simulink model "GFo_29bus"  (R2017b)
settings: Solver=ode1  StartTime=0.0  StopTime=4.5  FixedStep=Time_Step  RelTol=1e-3  EnableMultiTasking=on
PreLoadFcn:
  | Init_29bus;
InitFcn:
  | Init_29bus;
undefined symbols (not defined in the file): D1, D11, Delta, Time_Step, VSC01_Delta_P_Time_Step, VSC01_Delta_P_Value
libraries: powerlib x169, sps_avr x6, GFo_Lib x1
(part 2 of 5)

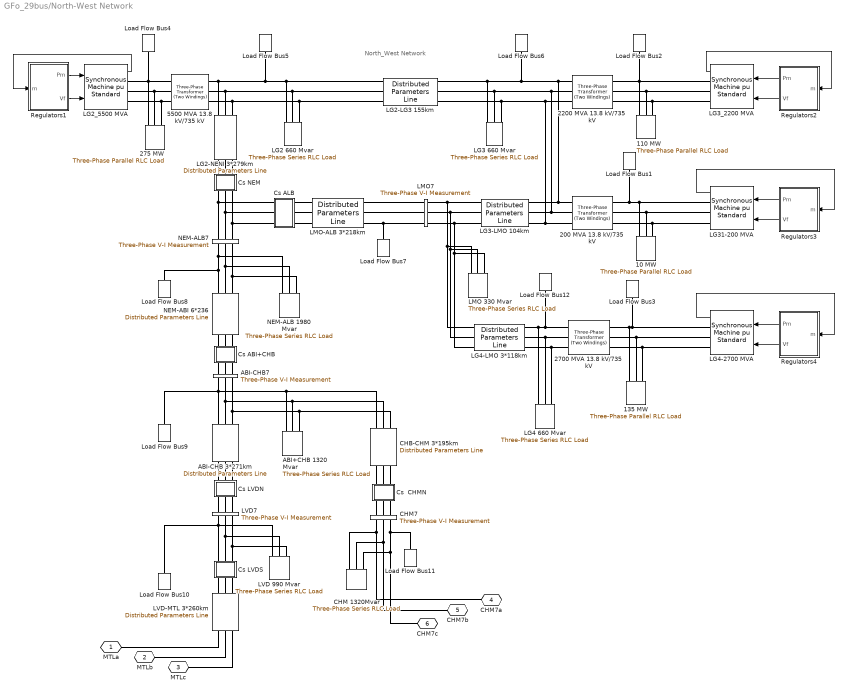
== system GFo_29bus/North-West Network ==
  note: North_West Network
  10 MW : powerlib/Elements/Three-Phase Parallel RLC Load  LConnTagsString=A|B|C  Configuration=Y (grounded)  NominalVoltage=(13800)*1  Vabc=[1e3 1e3 1e3]  Vabcp=[1e3 1e3 1e3]  NominalFrequency=60  UnbalancedPower=off  ActivePower=10000000  InductivePower=0  CapacitivePower=0  Pabc=[10e3 9e3 11e3]  QLabc=[100 90 110]  QCabc=[100 90 110]  Pabcp=[10e3 9e3 11e3]  QLabcp=[100 90 110]  QCabcp=[100 90 110]  Measurements=None  LoadType=constant PQ
  110 MW : powerlib/Elements/Three-Phase Parallel RLC Load  LConnTagsString=A|B|C  Configuration=Y (grounded)  NominalVoltage=(13800)*1  Vabc=[1e3 1e3 1e3]  Vabcp=[1e3 1e3 1e3]  NominalFrequency=60  UnbalancedPower=off  ActivePower=110000000  InductivePower=0  CapacitivePower=0  Pabc=[10e3 9e3 11e3]  QLabc=[100 90 110]  QCabc=[100 90 110]  Pabcp=[10e3 9e3 11e3]  QLabcp=[100 90 110]  QCabcp=[100 90 110]  Measurements=None  LoadType=constant PQ
  135 MW : powerlib/Elements/Three-Phase Parallel RLC Load  LConnTagsString=A|B|C  Configuration=Y (grounded)  NominalVoltage=(13800)*1  Vabc=[1e3 1e3 1e3]  Vabcp=[1e3 1e3 1e3]  NominalFrequency=60  UnbalancedPower=off  ActivePower=135000000  InductivePower=0  CapacitivePower=0  Pabc=[10e3 9e3 11e3]  QLabc=[100 90 110]  QCabc=[100 90 110]  Pabcp=[10e3 9e3 11e3]  QLabcp=[100 90 110]  QCabcp=[100 90 110]  Measurements=None  LoadType=constant PQ
  200 MVA 13.8 kV/735 kV : powerlib/Elements/Three-Phase Transformer (Two Windings)  Winding1Connection=Delta (D1)  Winding2Connection=Yg  CoreType=Three single-phase transformers  SetSaturation=off  Hysteresis=off  DataFile='basic_model'  SetInitialFlux=off  Measurements=None  UNITS=pu  NominalPower=[ 200e6 60 ]  Winding1="[ 13.8e3 0.002  0.0]"  Winding2=[ 735e3 0.002 0.12]  Rm=500  Lm=500  L0=0.5  Saturation="[ 0,0  ;  0.005,1.2  ;  1.0,1.4 ]"  InitialFluxes=[ 0.8 , -0.8 , 0.7 ]  BreakLoop=off  DiscreteSolver=Trapezoidal iterative  DataType=off  TransfoNumber=0
  2200 MVA 13.8 kV/735 kV : powerlib/Elements/Three-Phase Transformer (Two Windings)  Winding1Connection=Delta (D1)  Winding2Connection=Yg  CoreType=Three single-phase transformers  SetSaturation=off  Hysteresis=off  DataFile='basic_model'  SetInitialFlux=off  Measurements=None  UNITS=pu  NominalPower=[ 2200e6 60 ]  Winding1="[ 13.8e3 0.002  0.0]"  Winding2=[ 735e3 0.002 0.12]  Rm=500  Lm=500  L0=0.5  Saturation="[ 0,0  ;  0.005,1.2  ;  1.0,1.4 ]"  InitialFluxes=[ 0.8 , -0.8 , 0.7 ]  BreakLoop=off  DiscreteSolver=Trapezoidal iterative  DataType=off  TransfoNumber=0
  2700 MVA 13.8 kV/735 kV : powerlib/Elements/Three-Phase Transformer (Two Windings)  Winding1Connection=Delta (D1)  Winding2Connection=Yg  CoreType=Three single-phase transformers  SetSaturation=off  Hysteresis=off  DataFile='basic_model'  SetInitialFlux=off  Measurements=None  UNITS=pu  NominalPower=[ 2700e6 60 ]  Winding1="[ 13.8e3 0.002  0.0]"  Winding2=[ 735e3 0.002 0.12]  Rm=500  Lm=500  L0=0.5  Saturation="[ 0,0  ;  0.005,1.2  ;  1.0,1.4 ]"  InitialFluxes=[ 0.8 , -0.8 , 0.7 ]  BreakLoop=off  DiscreteSolver=Trapezoidal iterative  DataType=off  TransfoNumber=0
  275 MW : powerlib/Elements/Three-Phase Parallel RLC Load  LConnTagsString=A|B|C  Configuration=Y (grounded)  NominalVoltage=(13800)*1  Vabc=[1e3 1e3 1e3]  Vabcp=[1e3 1e3 1e3]  NominalFrequency=60  UnbalancedPower=off  ActivePower=275000000  InductivePower=0  CapacitivePower=0  Pabc=[10e3 9e3 11e3]  QLabc=[100 90 110]  QCabc=[100 90 110]  Pabcp=[10e3 9e3 11e3]  QLabcp=[100 90 110]  QCabcp=[100 90 110]  Measurements=None  LoadType=constant PQ
  5500 MVA 13.8 kV/735 kV : powerlib/Elements/Three-Phase Transformer (Two Windings)  Winding1Connection=Delta (D1)  Winding2Connection=Yg  CoreType=Three single-phase transformers  SetSaturation=off  Hysteresis=off  DataFile='basic_model'  SetInitialFlux=off  Measurements=None  UNITS=pu  NominalPower=[ 5500e6 60 ]  Winding1="[ 13.8e3 0.002  0.0]"  Winding2=[ 735e3 0.002 0.12]  Rm=500  Lm=500  L0=0.5  Saturation="[ 0,0  ;  0.005,1.2  ;  1.0,1.4 ]"  InitialFluxes=[ 0.8 , -0.8 , 0.7 ]  BreakLoop=off  DiscreteSolver=Trapezoidal iterative  DataType=off  TransfoNumber=0
  ABI+CHB 1320 Mvar : powerlib/Elements/Three-Phase Series RLC Load  LConnTagsString=A|B|C  Configuration=Y (grounded)  NominalVoltage=735e3  Vabc=[1e3 1e3 1e3]  Vabcp=[1e3 1e3 1e3]  NominalFrequency=60  UnbalancedPower=off  ActivePower=4400000  InductivePower=1320e6  CapacitivePower=0  Pabc=[10e3 9e3 11e3]  QLabc=[100 90 110]  QCabc=[100 90 110]  Pabcp=[10e3 9e3 11e3]  QLabcp=[100 90 110]  QCabcp=[100 90 110]  Measurements=None  LoadType=constant Z
  ABI-CHB 3*271km : powerlib/Elements/Distributed Parameters Line  Phases=3  Length=271  Frequency=60  Resistance="[0.01273  0.3864]/3"  Inductance="[0.9337e-3  4.1264e-3]/3"  Capacitance=[12.74e-9 7.751e-9]*3  x1=[-0.00156 -4.29903868088888e-08 0 0;-0.00152 -4.31049710047087e-08 0 0;-0.00148 -4.32097535018435e-08 0 0;-0.00144 -4.33047104736571e-08 0 0;-0.0014 -4.33898203277529e-08 0 0;-0.00136 -4.34650637108841e-08 0 0;-0.00132 -4.35304235133541e-08 0 0;-0.00128 -4.35858848729076e-08 0 0;-0.00124 -4.36314351781097e-08 0 0;-0.0012 -4.36670640712137e-08 0 0;-0.00116 -4.36927634505166e-08 0 0;-0.00112 -4.37085274722013e-08 0 0;-0.00108 -4.3714352551665e-08 0 0;-0.00104 -4.37102373643351e-08 0 0;-0.001 -4.36961828459695e-08 0 0;-0.00096 -4.36721921924446e-08 187826.147216155 -755236.018624265;-0.00092 -4.3638270859028e-08 199193.07837854 -752317.887920411;-0.00088 -4.35944265591385e-08 210514.71475267 -749228.686616557;-0.00084 -4.35406692625918e-08 221788.481896066 -745969.117170439;-0.0008 -4.34770111933336e-08 233011.816251302 -742539.920780041;-0.00076 -4.34034668266597e-08 244182.16572893 -738941.877215048;-0.00072 -4.3320052885925e-08 255296.99028781 -735175.804639541;-0.00068 -4.32267883387403e-08 266353.762512685 -731242.559425944;-0.00064 -4.31236943926593e-08 277349.968188901 -727143.035960301;-0.0006 -4.30107944903563e-08 288283.106874116 -722878.166438896;-0.00056 -4.28881143042955e-08 299150.692466876 -718448.920656278;-0.00052 -4.27556817308933e-08 309950.253771934 -713856.305784742;-0.00048 -4.26135268841747e-08 320679.335062181 -709101.366145305;-0.00044 -4.24616820889261e-08 331335.496637056 -704185.182970237;-0.0004 -4.23001818733444e-08 341916.315377312 -699108.874157196;-0.00036 -4.2129062961186e-08 352419.385296011 -693873.594015029;-0.00032 -4.19483642634157e-08 362842.318085629 -688480.533001295;-0.00028 -4.17581268693592e-08 373182.743661134 -682930.917451559;-0.00024 -4.15583940373594e-08 383438.310698921 -677226.00930054;-0.0002 -4.13492111849398e-08 393606.687171486 -671367.105795155;-0.00016 -4.11306258784772e-08 403685.560877708 -665355.539199535;-0.00012 -4.09026878223852e-08 413672.639968623 -659192.676492083;-8e-05 -4.06654488478122e-08 423565.653468569 -652879.919054632;-4e-05 -4.0418962900855e-08 433362.351791591 -646418.702353785]  x2=[-0.00156 -9.05659079389774e-08 0 0;-0.00152 -9.07557342875418e-08 0 0;-0.00148 -9.09249235647733e-08 0 0;-0.00144 -9.10734372984894e-08 0 0;-0.0014 -9.12012417179476e-08 0 0;-0.00136 -9.13083077615252e-08 0 0;-0.00132 -9.13946110833272e-08 0 0;-0.00128 -9.14601320587224e-08 0 0;-0.00124 -9.15048557888059e-08 0 0;-0.0012 -9.15287721037874e-08 0 0;-0.00116 -9.1531875565303e-08 0 0;-0.00112 -9.15141654676524e-08 0 0;-0.00108 -9.14756458379589e-08 0 0;-0.00104 -9.14163254352542e-08 0 0;-0.001 -9.13362177484864e-08 0 0;-0.00096 -9.12353409934526e-08 -41952.3785132872 -761003.958676694;-0.00092 -9.11137181086569e-08 -30472.3572703532 -761550.015312388;-0.00088 -9.09713767500946e-08 -18985.4068761582 -761922.902041928;-0.00084 -9.08083492849631e-08 -7494.13936416284 -762122.534074088;-0.0008 -9.0624672784302e-08 3998.83225049725 -762148.866014263;-0.00076 -9.04203890145636e-08 15490.8945651881 -762001.891874799;-0.00072 -9.01955444281156e-08 26979.4343840425 -761681.645076347;-0.00068 -8.99501901526778e-08 38461.8393121788 -761188.198440267;-0.00064 -8.96843819796967e-08 49935.4983497363 -760521.664172069;-0.0006 -8.93981803516586e-08 61397.8024855944 -759682.193835898;-0.00056 -8.90916503483457e-08 72846.1452906394 -758669.97832007;-0.00052 -8.87648616720371e-08 84277.9235104437 -757485.247793662;-0.00048 -8.84178886316599e-08 95690.5376572236 -756128.271654181;-0.00044 -8.80508101258913e-08 107081.39260094 -754599.358466298;-0.0004 -8.76637096252179e-08 118447.89815941 -752898.855891687;-0.00036 -8.72566751529554e-08 129787.46968729 -751027.15060997;-0.00032 -8.68297992652326e-08 141097.528663802 -748984.668230786;-0.00028 -8.63831790299452e-08 152375.503279069 -746771.873197016;-0.00024 -8.59169160046831e-08 163618.829018921 -744389.268679167;-0.0002 -8.54311162136376e-08 174824.949248043 -741837.39646096;-0.00016 -8.49258901234916e-08 185991.315791332 -739116.836816131;-0.00012 -8.44013526183013e-08 197115.38951333 -736228.208376482;-8e-05 -8.38576229733718e-08 208194.640895605 -733172.16799121;-4e-05 -8.32948248281354e-08 219226.550611933 -729949.410577544]  x3=[-0.00156 -1.87807393079567e-10 0 0;-0.00152 -1.93846462957491e-10 0 0;-0.00148 -1.998414538214e-10 0 0;-0.00144 -2.05791002462069e-10 0 0;-0.0014 -2.11693756003443e-10 0 0;-0.00136 -2.17548372210272e-10 0 0;-0.00132 -2.23353519793318e-10 0 0;-0.00128 -2.29107878712081e-10 0 0;-0.00124 -2.34810140474967e-10 0 0;-0.0012 -2.40459008436826e-10 0 0;-0.00116 -2.46053198093796e-10 0 0;-0.00112 -2.51591437375393e-10 0 0;-0.00108 -2.57072466933762e-10 0 0;-0.00104 -2.62495040430049e-10 0 0;-0.001 -2.67857924817803e-10 0 0;-0.00096 -2.73159900623362e-10 139.26170460855 -1341.51413253579;-0.00092 -2.78399762223149e-10 159.474777343631 -1339.26171709775;-0.00088 -2.83576318117825e-10 179.651586889596 -1336.70476509455;-0.00084 -2.88688391203218e-10 199.787545213952 -1333.84385795502;-0.0008 -2.93734819037995e-10 219.87807357342 -1330.67964622477;-0.00076 -2.98714454107983e-10 239.918603555106 -1327.21284941825;-0.00072 -3.03626164087111e-10 259.904578115313 -1323.44425585518;-0.00068 -3.08468832094887e-10 279.831452615779 -1319.37472248122;-0.00064 -3.13241356950365e-10 299.694695857083 -1315.00517467318;-0.0006 -3.17942653422552e-10 319.489791109006 -1310.33660602853;-0.00056 -3.22571652477171e-10 339.212237137594 -1305.37007813954;-0.00052 -3.27127301519756e-10 358.857549228699 -1300.10672035181;-0.00048 -3.31608564635002e-10 378.421260207764 -1294.54772950751;-0.00044 -3.36014422822319e-10 397.898921455624 -1288.69436967323;-0.0004 -3.40343874227552e-10 417.28610392008 -1282.54797185251;-0.00036 -3.44595934370786e-10 436.578399123026 -1276.10993368321;-0.00032 -3.48769636370213e-10 455.771420162903 -1269.3817191197;-0.00028 -3.52864031161991e-10 474.86080271224 -1262.36485809994;-0.00024 -3.56878187716052e-10 493.842206010066 -1255.06094619762;-0.0002 -3.60811193247813e-10 512.711313848959 -1247.47164425932;-0.00016 -3.64662153425733e-10 531.463835556517 -1239.59867802686;-0.00012 -3.68430192574676e-10 550.095506971018 -1231.44383774485;-8e-05 -3.72114453875034e-10 568.602091411056 -1223.00897775366;-4e-05 -3.7571409955756e-10 586.979380638922 -1214.29601606771]  x4=[-0.00156 -2.85151300335962e-10 0 0;-0.00152 -2.82558887702488e-10 0 0;-0.00148 -2.79902223614635e-10 0 0;-0.00144 -2.77181912174905e-10 0 0;-0.0014 -2.74398571958662e-10 0 0;-0.00136 -2.71552835873468e-10 0 0;-0.00132 -2.68645351015168e-10 0 0;-0.00128 -2.65676778520747e-10 0 0;-0.00124 -2.62647793417989e-10 0 0;-0.0012 -2.59559084471985e-10 0 0;-0.00116 -2.56411354028515e-10 0 0;-0.00112 -2.53205317854336e-10 0 0;-0.00108 -2.49941704974427e-10 0 0;-0.00104 -2.46621257506212e-10 0 0;-0.001 -2.43244730490811e-10 0 0;-0.00096 -2.3981289172135e-10 -1510.55195138726 -15585.3803111079;-0.00092 -2.36326521568369e-10 -1275.36683491832 -15606.38544091;-0.00088 -2.32786412802377e-10 -1039.89171102942 -15623.8418132467;-0.00084 -2.29193370413579e-10 -804.180124733081 -15637.7454586893;-0.0008 -2.25548211428828e-10 -568.285674811329 -15648.0932156687;-0.00076 -2.21851764725842e-10 -332.262001627809 -15654.8827311943;-0.00072 -2.18104870844727e-10 -96.1627749304264 -15658.1124613888;-0.00068 -2.14308381796837e-10 139.958318352703 -15657.7816718394;-0.00064 -2.10463160871044e-10 376.047586321189 -15653.8904377648;-0.0006 -2.06570082437426e-10 612.051344311441 -15646.439643998;-0.00056 -2.02630031748445e-10 847.915927104103 -15635.4309847854;-0.00052 -1.98643904737653e-10 1083.58770112706 -15620.866963401;-0.00048 -1.94612607815955e-10 1319.01307665124 -15602.7508915777;-0.00044 -1.90537057665507e-10 1554.13851997647 -15581.0868887541;-0.0004 -1.86418181031268e-10 1788.91056560458 -15555.8798811376;-0.00036 -1.82256914510264e-10 2023.27582839698 -15527.1356005843;-0.00032 -1.78054204338617e-10 2257.18101571399 -15494.8605832957;-0.00028 -1.73811006176378e-10 2490.57293953313 -15459.0621683325;-0.00024 -1.69528284890216e-10 2723.3985285436 -15419.7484959455;-0.0002 -1.6520701433402e-10 2955.60484021427 -15376.9285057247;-0.00016 -1.60848177127449e-10 3187.13907283233 -15330.6119345667;-0.00012 -1.56452764432495e-10 3417.94857750994 -15280.8093144604;-8e-05 -1.520217757281e-10 3647.98087015616 -15227.531970092;-4e-05 -1.47556218582885e-10 3877.18364341136 -15170.7920162703]  x5=0.00153261764655846  V1=ones(3,3)  V2=ones(3,3)  I1=ones(3,3)  I2=ones(3,3)  nHarmo=1  Measurements=None  Decoupling=off  VsMag0=0  VrMag0=0  VsAngle0=0  VrAngle0=0  IsMag0=0  IrMag0=0  IsAngle0=0  IrAngle0=0
      settings: AttributesFormatString=\n
  ABI-CHB7 : powerlib/Measurements/Three-Phase V-I Measurement  VoltageMeasurement=no  SetLabelV=on  LabelV=Vabc_ABI7  Vpu=on  VpuLL=off  CurrentMeasurement=no  SetLabelI=off  LabelI=A1  Ipu=off  Pbase=100e6  Vbase=500e3  OutputType=Magnitude  PhasorSimulation=off  PSBequivalent=0
  CHB-CHM 3*195km : powerlib/Elements/Distributed Parameters Line  Phases=3  Length=195  Frequency=60  Resistance="[0.01273  0.3864]/3"  Inductance="[0.9337e-3  4.1264e-3]/3"  Capacitance=[12.74e-9 7.751e-9]*3  x1=[-0.00112 -4.32880028151544e-08 0 0;-0.00108 -4.32972814037169e-08 0 0;-0.00104 -4.32967145638679e-08 0 0;-0.001 -4.32863024245021e-08 0 0;-0.00096 -4.32660473532502e-08 0 0;-0.00092 -4.32359539559406e-08 0 0;-0.00088 -4.31960290755524e-08 0 0;-0.00084 -4.31462817906592e-08 0 0;-0.0008 -4.30867234133644e-08 0 0;-0.00076 -4.30173674867295e-08 0 0;-0.00072 -4.29382297816941e-08 0 0;-0.00068 -4.28493282934899e-08 266353.762512684 -731242.559425945;-0.00064 -4.27506832375486e-08 277349.968188901 -727143.035960302;-0.0006 -4.26423170449053e-08 288283.106874116 -722878.166438896;-0.00056 -4.25242543570976e-08 299150.692466875 -718448.920656278;-0.00052 -4.23965220205627e-08 309950.253771933 -713856.305784743;-0.00048 -4.22591490805323e-08 320679.335062181 -709101.366145306;-0.00044 -4.21121667744285e-08 331335.496637056 -704185.182970238;-0.0004 -4.19556085247599e-08 341916.315377311 -699108.874157197;-0.00036 -4.17895099315226e-08 352419.385296011 -693873.59401503;-0.00032 -4.16139087641043e-08 362842.318085629 -688480.533001296;-0.00028 -4.1428844952696e-08 373182.743661134 -682930.91745156;-0.00024 -4.12343605792127e-08 383438.310698921 -677226.009300541;-0.0002 -4.10304998677236e-08 393606.687171486 -671367.105795156;-0.00016 -4.08173091743966e-08 403685.560877708 -665355.539199536;-0.00012 -4.05948369769568e-08 413672.639968622 -659192.676492084;-8e-05 -4.03631338636634e-08 423565.653468569 -652879.919054633;-4e-05 -4.01222525218062e-08 433362.351791591 -646418.702353786]  x2=[-0.00112 -3.01476576023589e-08 0 0;-0.00108 -3.01218550239861e-08 0 0;-0.00104 -3.00892029955408e-08 0 0;-0.001 -3.00497089418125e-08 0 0;-0.00096 -3.00033818434085e-08 0 0;-0.00092 -2.99502322347114e-08 0 0;-0.00088 -2.9890272201484e-08 0 0;-0.00084 -2.98235153781207e-08 0 0;-0.0008 -2.97499769445474e-08 0 0;-0.00076 -2.96696736227698e-08 0 0;-0.00072 -2.95826236730708e-08 0 0;-0.00068 -2.94888468898582e-08 189059.279164108 -739106.876621136;-0.00064 -2.93883645971639e-08 200182.856377785 -736171.980404537;-0.0006 -2.92811996437946e-08 211260.913736226 -733069.685028072;-0.00056 -2.91673763981366e-08 222290.93218472 -729800.695926955;-0.00052 -2.90469207426144e-08 233270.40359219 -726365.756441117;-0.00048 -2.89198600678053e-08 244196.831321521 -722765.647646176;-0.00044 -2.87862232662111e-08 255067.730797274 -719001.188175825;-0.0004 -2.86460407256879e-08 265880.630070654 -715073.234035686;-0.00036 -2.84993443225366e-08 276633.070381613 -710982.678408656;-0.00032 -2.83461674142543e-08 287322.606717949 -706730.451451809;-0.00028 -2.81865448319489e-08 297946.808371282 -702317.520084886;-0.00024 -2.80205128724192e-08 308503.259489775 -697744.887770424;-0.0002 -2.78481092899009e-08 318989.559627479 -693013.594285579;-0.00016 -2.76693732874819e-08 329403.324290172 -688124.715485687;-0.00012 -2.74843455081878e-08 339742.185477576 -683079.36305963;-8e-05 -2.72930680257401e-08 350003.792221813 -677878.684277038;-4e-05 -2.70955843349887e-08 360185.811122003 -672523.861727418]  x3=[-0.00112 -1.55990618873976e-10 0 0;-0.00108 -1.5474156304947e-10 0 0;-0.00104 -1.5345732032796e-10 0 0;-0.001 -1.52138182735167e-10 0 0;-0.00096 -1.50784450231604e-10 0 0;-0.00092 -1.49396430644368e-10 0 0;-0.00088 -1.47974439597144e-10 0 0;-0.00084 -1.46518800438432e-10 0 0;-0.0008 -1.45029844168025e-10 0 0;-0.00076 -1.43507909361738e-10 0 0;-0.00072 -1.41953342094422e-10 0 0;-0.00068 -1.40366495861267e-10 1436.68883540973 -5039.584986483;-0.00064 -1.38747731497423e-10 1512.51770857072 -5017.34797479882;-0.0006 -1.37097417095945e-10 1588.00264824819 -4993.97006145294;-0.00056 -1.35415927924098e-10 1663.1264898178 -4969.45656238125;-0.00052 -1.33703646338018e-10 1737.87215076581 -4943.81305174204;-0.00048 -1.31960961695771e-10 1812.22263457351 -4917.04536064849;-0.00044 -1.30188270268818e-10 1886.16103458205 -4889.15957584272;-0.0004 -1.28385975151902e-10 1959.67053783689 -4860.16203831173;-0.00036 -1.26554486171389e-10 2032.7344289109 -4830.05934184547;-0.00032 -1.24694219792081e-10 2105.33609370534 -4798.85833153754;-0.00028 -1.22805599022509e-10 2177.45902322771 -4766.56610222861;-0.00024 -1.2088905331875e-10 2249.0868173458 -4733.18999689314;-0.0002 -1.18945018486769e-10 2320.20318851693 -4698.73760496967;-0.00016 -1.16973936583322e-10 2390.79196549157 -4663.21676063503;-0.00012 -1.14976255815436e-10 2460.83709699057 -4626.63554102288;-8e-05 -1.12952430438491e-10 2530.32265535507 -4589.00226438711;-4e-05 -1.10902920652924e-10 2599.23284016831 -4550.32548821028]  x4=[-0.00112 -1.20875953871152e-10 0 0;-0.00108 -1.23066019964183e-10 0 0;-0.00104 -1.25228101905551e-10 0 0;-0.001 -1.27361708056466e-10 0 0;-0.00096 -1.2946635325329e-10 0 0;-0.00092 -1.31541558917854e-10 0 0;-0.00088 -1.33586853166286e-10 0 0;-0.00084 -1.35601770916312e-10 0 0;-0.0008 -1.37585853993012e-10 0 0;-0.00076 -1.39538651233004e-10 0 0;-0.00072 -1.41459718587035e-10 0 0;-0.00068 -1.43348619220956e-10 1508.00651437468 -11782.2938614793;-0.00064 -1.45204923615053e-10 1685.50172841821 -11758.214496796;-0.0006 -1.47028209661713e-10 1862.61367390384 -11731.4614155346;-0.00056 -1.48818062761413e-10 2039.30207710253 -11702.0407011152;-0.00052 -1.50574075916994e-10 2215.52676059507 -11669.9590435544;-0.00048 -1.52295849826207e-10 2391.24765240814 -11635.2237379446;-0.00044 -1.53982992972513e-10 2566.4247951263 -11597.8426827946;-0.0004 -1.55635121714109e-10 2741.01835497795 -11557.8243782342;-0.00036 -1.57251860371168e-10 2914.98863089321 -11515.1779240805;-0.00032 -1.58832841311261e-10 3088.2960635316 -11469.9130177696;-0.00028 -1.60377705032956e-10 3260.90124427747 -11422.0399521507;-0.00024 -1.61886100247564e-10 3432.76492420121 -11371.5696131462;-0.0002 -1.63357683959023e-10 3603.84802298409 -11318.513477276;-0.00016 -1.64792121541886e-10 3774.1116378048 -11262.8836090476;-0.00012 -1.66189086817417e-10 3943.51705218563 -11204.6926582136;-8e-05 -1.67548262127759e-10 4112.02574479624 -11143.9538568943;-4e-05 -1.68869338408169e-10 4279.59939821308 -11080.6810165692]  x5=0.0011028060556417  V1=ones(3,3)  V2=ones(3,3)  I1=ones(3,3)  I2=ones(3,3)  nHarmo=1  Measurements=None  Decoupling=off  VsMag0=0  VrMag0=0  VsAngle0=0  VrAngle0=0  IsMag0=0  IrMag0=0  IsAngle0=0  IrAngle0=0
      settings: AttributesFormatString=\n
  CHM 1320Mvar : powerlib/Elements/Three-Phase Series RLC Load  LConnTagsString=A|B|C  Configuration=Y (grounded)  NominalVoltage=735e3  Vabc=[1e3 1e3 1e3]  Vabcp=[1e3 1e3 1e3]  NominalFrequency=60  UnbalancedPower=off  ActivePower=4400000  InductivePower=1320e6  CapacitivePower=0  Pabc=[10e3 9e3 11e3]  QLabc=[100 90 110]  QCabc=[100 90 110]  Pabcp=[10e3 9e3 11e3]  QLabcp=[100 90 110]  QCabcp=[100 90 110]  Measurements=None  LoadType=constant Z
  CHM7 : powerlib/Measurements/Three-Phase V-I Measurement  VoltageMeasurement=no  SetLabelV=on  LabelV=Vabc_CHM7  Vpu=on  VpuLL=off  CurrentMeasurement=no  SetLabelI=off  LabelI=A1  Ipu=off  Pbase=100e6  Vbase=735e3  OutputType=Magnitude  PhasorSimulation=off  PSBequivalent=0
  "Cs  CHMN " : Subsystem  mask{Xc=25/3}
      mask prompts: Xc "Condensator Reactance at  60Hz  (ohm):"
      mask help: Series Compensation
      mask init:
      | Cs=1/Xc/(2*pi*60);
      mask Display: disp('Cs')
  "Cs ABI+CHB " : Subsystem  mask{Xc=25/6}
      mask prompts: Xc "Condensator Reactance at  60Hz  (ohm):"
      mask help: Series Compensation
      mask init:
      | Cs=1/Xc/(2*pi*60);
      mask Display: disp('Cs')
  Cs ALB : Subsystem  mask{Xc=16/3}
      mask prompts: Xc "Reactance @ 60Hz du condensateur (ohm):"
      mask init:
      | Cs=1/Xc/(2*pi*60);
      mask Display: disp('Cs')
  "Cs LVDN " : Subsystem  mask{Xc=34/3}
      mask prompts: Xc "Condensator Reactance at  60Hz  (ohm):"
      mask help: Series Compensation
      mask init:
      | Cs=1/Xc/(2*pi*60);
      mask Display: disp('Cs')
  "Cs LVDS " : Subsystem  mask{Xc=34/3}
      mask prompts: Xc "Condensator Reactance at  60Hz  (ohm):"
      mask help: Series Compensation
      mask init:
      | Cs=1/Xc/(2*pi*60);
      mask Display: disp('Cs')
  "Cs NEM " : Subsystem  mask{Xc=16/3}
      mask prompts: Xc "Condensator Reactance at  60Hz  (ohm):"
      mask help: Series Compensation
      mask init:
      | Cs=1/Xc/(2*pi*60);
      mask Display: disp('Cs')
  LG2 660 Mvar : powerlib/Elements/Three-Phase Series RLC Load  LConnTagsString=A|B|C  Configuration=Y (grounded)  NominalVoltage=735e3  Vabc=[1e3 1e3 1e3]  Vabcp=[1e3 1e3 1e3]  NominalFrequency=60  UnbalancedPower=off  ActivePower=2200000  InductivePower=660e6  CapacitivePower=0  Pabc=[10e3 9e3 11e3]  QLabc=[100 90 110]  QCabc=[100 90 110]  Pabcp=[10e3 9e3 11e3]  QLabcp=[100 90 110]  QCabcp=[100 90 110]  Measurements=None  LoadType=constant Z
  LG2-LG3 155km : powerlib/Elements/Distributed Parameters Line  Phases=3  Length=155  Frequency=60  Resistance="[0.01273  0.3864]"  Inductance="[0.9337e-3  4.1264e-3]"  Capacitance=[12.74e-9 7.751e-9]  x1=[-0.00088 -2.79013421874721e-09 432972.643007631 -601762.460463105;-0.00084 -2.80512262966329e-09 441997.469610389 -595165.210789451;-0.0008 -2.81947317988372e-09 450921.789800182 -588432.625679351;-0.00076 -2.83318260621716e-09 459743.574263559 -581566.236064597;-0.00072 -2.84624779125826e-09 468460.817002808 -574567.603302976;-0.00068 -2.85866576409663e-09 477071.535792104 -567438.318823225;-0.00064 -2.87043370099233e-09 485573.772628251 -560180.003763152;-0.0006 -2.88154892601799e-09 493965.594175912 -552794.30860101;-0.00056 -2.89200891166729e-09 502245.092207235 -545282.912780187;-0.00052 -2.9018112794297e-09 510410.384035767 -537647.524327318;-0.00048 -2.91095380033132e-09 518459.612944562 -529889.879463891;-0.00044 -2.91943439544175e-09 526390.948608378 -522011.742211451;-0.0004 -2.92725113634678e-09 534202.587509883 -514014.903990468;-0.00036 -2.93440224558694e-09 541892.753349755 -505901.183212994;-0.00032 -2.94088609706166e-09 549459.697450599 -497672.424869164;-0.00028 -2.94670121639904e-09 556901.699154582 -489330.500107662;-0.00024 -2.95184628129107e-09 564217.066214693 -480877.305810242;-0.0002 -2.95632012179438e-09 571404.135179547 -472314.764160391;-0.00016 -2.96012172059621e-09 578461.271771641 -463644.822206238;-0.00012 -2.96325021324578e-09 585386.871258971 -454869.451417819;-8e-05 -2.96570488835083e-09 592179.358819939 -445990.647238774;-4e-05 -2.96748518773943e-09 598837.189901448 -437010.428632606]  x2=[-0.00088 -1.73659978268186e-09 445028.99986202 -584528.468417321;-0.00084 -1.75470646929317e-09 453792.58140898 -577751.376044598;-0.0008 -1.77241415078531e-09 462452.974436268 -570842.907991278;-0.00076 -1.78971880058422e-09 471008.209645194 -563804.635183421;-0.00072 -1.80661648376174e-09 479456.341649048 -556638.158063567;-0.00068 -1.82310335793046e-09 487795.449415467 -549345.106226812;-0.00064 -1.83917567411735e-09 496023.636703258 -541927.138050252;-0.0006 -1.85482977761633e-09 504139.032493588 -534385.94031588;-0.00056 -1.87006210881925e-09 512139.791415439 -526723.227827028;-0.00052 -1.88486920402535e-09 520024.094165227 -518940.743018436;-0.00048 -1.89924769622888e-09 527790.147920499 -511040.255560035;-0.00044 -1.9131943158847e-09 535436.186747602 -503023.561954544;-0.0004 -1.92670589165177e-09 542960.472003244 -494892.485128955;-0.00036 -1.93977935111428e-09 550361.292729844 -486648.874020019;-0.00032 -1.95241172148029e-09 557636.96604459 -478294.603153812;-0.00028 -1.96460013025773e-09 564785.837522115 -469831.572219484;-0.00024 -1.97634180590753e-09 571806.281570693 -461261.705637289;-0.0002 -1.98763407847391e-09 578696.701801889 -452586.952120983;-0.00016 -1.99847438019147e-09 585455.531393563 -443809.284234708;-0.00012 -2.00886024606909e-09 592081.233446151 -434930.697944447;-8e-05 -2.01878931445043e-09 598572.301332146 -425953.212164156;-4e-05 -2.02825932755095e-09 604927.259038684 -416878.868296683]  x3=[-0.00088 -1.84558852963393e-12 1691.06014924484 -2581.83555987813;-0.00084 -1.82016083348527e-12 1729.79962719175 -2556.042391552;-0.0008 -1.79431924845947e-12 1768.1457636206 -2529.66800122839;-0.00076 -1.76806965071012e-12 1806.08983895064 -2502.71838621624;-0.00072 -1.74141800916939e-12 1843.62322502635 -2475.19967462559;-0.00068 -1.71437038419072e-12 1880.73738707943 -2447.11812397413;-0.00064 -1.68693292617078e-12 1917.42388566947 -2418.48011976434;-0.0006 -1.65911187415093e-12 1953.67437860307 -2389.29217403139;-0.00056 -1.63091355439846e-12 1989.48062283075 -2359.56092386245;-0.00052 -1.60234437896812e-12 2024.83447632134 -2329.29312988741;-0.00048 -1.57341084424404e-12 2059.72789991345 -2298.4956747416;-0.00044 -1.54411952946249e-12 2094.15295914345 -2267.17556150074;-0.0004 -1.51447709521586e-12 2128.10182604975 -2235.33991208848;-0.00036 -1.48449028193807e-12 2161.56678095278 -2202.99596565696;-0.00032 -1.45416590837187e-12 2194.54021421037 -2170.15107694068;-0.00028 -1.4235108700183e-12 2227.01462794816 -2136.81271458409;-0.00024 -1.39253213756872e-12 2258.98263776451 -2102.98845944329;-0.0002 -1.36123675531974e-12 2290.43697440968 -2068.68600286221;-0.00016 -1.32963183957141e-12 2321.37048543874 -2033.91314492367;-0.00012 -1.29772457700902e-12 2351.77613683807 -1998.6777926757;-8e-05 -1.26552222306891e-12 2381.64701462473 -1962.98795833353;-4e-05 -1.23303210028868e-12 2410.97632641872 -1926.85175745773]  x4=[-0.00088 -4.62619871537164e-12 1092.96989342995 -2102.93040181752;-0.00084 -4.72627398977189e-12 1124.55604688283 -2086.21026082643;-0.0008 -4.82527455022451e-12 1155.8864859884 -2069.01573361274;-0.00076 -4.92317788485581e-12 1186.95408647501 -2051.35073006366;-0.00072 -5.01996173129177e-12 1217.7517838382 -2033.21926704865;-0.00068 -5.11560408172034e-12 1248.2725749472 -2014.62546750606;-0.00064 -5.21008318789582e-12 1278.50951963729 -1995.57355950554;-0.0006 -5.30337756608421e-12 1308.45574228802 -1976.06787528669;-0.00056 -5.39546600194846e-12 1338.10443338659 -1956.11285027387;-0.00052 -5.48632755537238e-12 1367.44885107633 -1935.71302206771;-0.00048 -5.57594156522228e-12 1396.48232268971 -1914.8730294132;-0.00044 -5.66428765404513e-12 1425.19824626567 -1893.59761114497;-0.0004 -5.75134573270218e-12 1453.59009205081 -1871.89160510966;-0.00036 -5.83709600493711e-12 1481.65140398424 -1849.75994706585;-0.00032 -5.92151897187748e-12 1509.37580116563 -1827.20766956172;-0.00028 -6.00459543646866e-12 1536.75697930613 -1804.23990079071;-0.00024 -6.08630650783901e-12 1563.78871216196 -1780.86186342535;-0.0002 -6.16663360559555e-12 1590.46485295019 -1757.07887342976;-0.00016 -6.24555846404895e-12 1616.77933574645 -1732.89633885075;-0.00012 -6.32306313636704e-12 1642.72617686427 -1708.31975858814;-8e-05 -6.39912999865569e-12 1668.29947621573 -1683.35472114436;-4e-05 -6.4737417539664e-12 1693.49341865311 -1658.00690335361]  x5=0.000876589428843401  V1=ones(3,3)  V2=ones(3,3)  I1=ones(3,3)  I2=ones(3,3)  nHarmo=1  Measurements=None  Decoupling=off  VsMag0=0  VrMag0=0  VsAngle0=0  VrAngle0=0  IsMag0=0  IrMag0=0  IsAngle0=0  IrAngle0=0
      settings: AttributesFormatString=\n
  LG2-NENI 3*279km : powerlib/Elements/Distributed Parameters Line  Phases=3  Length=279  Frequency=60  Resistance="[0.01273  0.3864]/3"  Inductance="[0.9337e-3  4.1264e-3]/3"  Capacitance=[12.74e-9 7.751e-9]*3  x1=[-0.0016 -2.41583924208325e-09 0 0;-0.00156 -2.4415900454317e-09 0 0;-0.00152 -2.46678565225921e-09 0 0;-0.00148 -2.49142033330204e-09 0 0;-0.00144 -2.51548848684617e-09 0 0;-0.0014 -2.53898464000105e-09 0 0;-0.00136 -2.56190344994405e-09 0 0;-0.00132 -2.58423970513546e-09 0 0;-0.00128 -2.60598832650345e-09 0 0;-0.00124 -2.62714436859908e-09 0 0;-0.0012 -2.64770302072082e-09 0 0;-0.00116 -2.66765960800847e-09 0 0;-0.00112 -2.68700959250617e-09 0 0;-0.00108 -2.70574857419432e-09 0 0;-0.00104 -2.72387229199008e-09 0 0;-0.001 -2.74137662471631e-09 405315.757865484 -620727.351198764;-0.00096 -2.75825759203871e-09 414629.701621834 -614544.98398557;-0.00092 -2.77451135537088e-09 423849.362159649 -608222.874542627;-0.00088 -2.79013421874721e-09 432972.643007631 -601762.460463105;-0.00084 -2.80512262966329e-09 441997.469610389 -595165.210789451;-0.0008 -2.81947317988372e-09 450921.789800182 -588432.625679351;-0.00076 -2.83318260621716e-09 459743.574263559 -581566.236064597;-0.00072 -2.84624779125826e-09 468460.817002808 -574567.603302976;-0.00068 -2.85866576409663e-09 477071.535792104 -567438.318823225;-0.00064 -2.87043370099233e-09 485573.772628251 -560180.003763152;-0.0006 -2.88154892601799e-09 493965.594175912 -552794.30860101;-0.00056 -2.89200891166729e-09 502245.092207235 -545282.912780187;-0.00052 -2.9018112794297e-09 510410.384035767 -537647.524327318;-0.00048 -2.91095380033132e-09 518459.612944562 -529889.879463891;-0.00044 -2.91943439544175e-09 526390.948608378 -522011.742211451;-0.0004 -2.92725113634678e-09 534202.587509883 -514014.903990468;-0.00036 -2.93440224558694e-09 541892.753349755 -505901.183212994;-0.00032 -2.94088609706166e-09 549459.697450599 -497672.424869164;-0.00028 -2.94670121639904e-09 556901.699154582 -489330.500107662;-0.00024 -2.95184628129107e-09 564217.066214693 -480877.305810242;-0.0002 -2.95632012179438e-09 571404.135179547 -472314.764160391;-0.00016 -2.96012172059621e-09 578461.271771641 -463644.822206238;-0.00012 -2.96325021324578e-09 585386.871258971 -454869.451417819;-8e-05 -2.96570488835083e-09 592179.358819939 -445990.647238774;-4e-05 -2.96748518773943e-09 598837.189901448 -437010.428632606]  x2=[-0.0016 -2.65953235838337e-08 0 0;-0.00156 -2.66692370020041e-08 0 0;-0.00152 -2.6737086065666e-08 0 0;-0.00148 -2.67988553465273e-08 0 0;-0.00144 -2.68545307987864e-08 0 0;-0.0014 -2.69040997623254e-08 0 0;-0.00136 -2.69475509655895e-08 0 0;-0.00132 -2.69848745281498e-08 0 0;-0.00128 -2.70160619629501e-08 0 0;-0.00124 -2.70411061782365e-08 0 0;-0.0012 -2.70600014791707e-08 0 0;-0.00116 -2.70727435691239e-08 0 0;-0.00112 -2.7079329550655e-08 0 0;-0.00108 -2.70797579261684e-08 0 0;-0.00104 -2.70740285982553e-08 0 0;-0.001 -2.70621428697155e-08 243862.200065526 -727663.308973734;-0.00096 -2.7044103443261e-08 254806.991474596 -723903.345217305;-0.00092 -2.7019914420902e-08 265693.841971167 -719978.77208285;-0.00088 -2.69895813030134e-08 276520.27597932 -715890.481984456;-0.00084 -2.69531109870848e-08 287283.831661325 -711639.404564035;-0.0008 -2.69105117661515e-08 297982.06147744 -707226.506479933;-0.00076 -2.68617933269089e-08 308612.532742463 -702652.79118712;-0.00072 -2.680696674751e-08 319172.828178901 -697919.29870901;-0.00068 -2.67460444950462e-08 329660.54646664 -693027.105400973;-0.00064 -2.66790404227122e-08 340073.302788985 -687977.323705579;-0.0006 -2.66059697666564e-08 350408.729374943 -682771.101899639;-0.00056 -2.65268491425158e-08 360664.476037637 -677409.623833093;-0.00052 -2.64416965416379e-08 370838.210708718 -671894.10865982;-0.00048 -2.635053132699e-08 380927.619968656 -666225.810560406;-0.00044 -2.62533742287556e-08 390930.409572794 -660406.018456956;-0.0004 -2.6150247339621e-08 400844.304973034 -654436.055720009;-0.00036 -2.60411741097515e-08 410667.051835058 -648317.279867607;-0.00032 -2.59261793414591e-08 420396.416550937 -642051.082256614;-0.00028 -2.58052891835622e-08 430030.186747036 -635638.887766327;-0.00024 -2.56785311254403e-08 439566.171787091 -629082.15447448;-0.0002 -2.55459339907826e-08 449002.203270339 -622382.373325678;-0.00016 -2.54075279310343e-08 458336.135524594 -615541.067792378;-0.00012 -2.52633444185396e-08 467565.846094152 -608559.793528464;-8e-05 -2.51134162393859e-08 476689.236222426 -601440.138015496;-4e-05 -2.49577774859483e-08 485704.231329174 -594183.720201743]  x3=[-0.0016 -1.94345070726738e-11 0 0;-0.00156 -2.20044197367152e-11 0 0;-0.00152 -2.45693287854664e-11 0 0;-0.00148 -2.71286509807287e-11 0 0;-0.00144 -2.96818043547055e-11 0 0;-0.0014 -3.2228208342337e-11 0 0;-0.00136 -3.47672839133157e-11 0 0;-0.00132 -3.72984537037529e-11 0 0;-0.00128 -3.98211421474659e-11 0 0;-0.00124 -4.23347756068575e-11 0 0;-0.0012 -4.48387825033557e-11 0 0;-0.00116 -4.73325934473858e-11 0 0;-0.00112 -4.98156413678448e-11 0 0;-0.00108 -5.22873616410486e-11 0 0;-0.00104 -5.47471922191222e-11 0 0;-0.001 -5.7194573757805e-11 -295.463539845799 -2742.88515404389;-0.00096 -5.96289497436401e-11 -254.069695761354 -2747.02858680455;-0.00092 -6.20497666205217e-11 -212.618078419097 -2750.54736895394;-0.00088 -6.44564739155682e-11 -171.118113559348 -2753.44070035133;-0.00084 -6.68485243642953e-11 -129.579237916235 -2755.70792307813;-0.0008 -6.9225374035059e-11 -88.0108970718639 -2757.34852158744;-0.00076 -7.15864824527414e-11 -46.4225433084721 -2758.3621228213;-0.00072 -7.39313127216495e-11 -4.823633459063 -2758.74849629552;-0.00068 -7.62593316476013e-11 36.7763732429975 -2758.50755415213;-0.00064 -7.85700098591688e-11 78.3680173149285 -2757.63935117928;-0.0006 -8.08628219280533e-11 119.941841175539 -2756.14408479883;-0.00056 -8.31372464885626e-11 161.488391295801 -2754.02209502148;-0.00052 -8.53927663561655e-11 202.998220348498 -2751.2738643694;-0.00048 -8.76288686450949e-11 244.461889356471 -2747.90001776653;-0.00044 -8.98450448849735e-11 285.869969838953 -2743.9013223965;-0.0004 -9.2040791136436e-11 327.213045955531 -2739.27868752816;-0.00036 -9.421560810572e-11 368.481716647225 -2734.03316430881;-0.00032 -9.63690012582015e-11 409.666597774204 -2728.16594552519;-0.00028 -9.85004809308479e-11 450.758324249663 -2721.67836533226;-0.00024 -1.00609562443563e-10 491.747552169362 -2714.57189894981;-0.0002 -1.02695766209397e-10 532.624960936348 -2706.84816232701;-0.00016 -1.04758617843607e-10 573.381255380379 -2698.50891177496;-0.00012 -1.06797648271518e-10 614.007167871566 -2689.55604356732;-8e-05 -1.08812393835197e-10 654.493460427751 -2679.99159350911;-4e-05 -1.10802396398875e-10 694.830926815146 -2669.81773647381]  x4=[-0.0016 -7.71465364255446e-11 0 0;-0.00156 -7.54489471332153e-11 0 0;-0.00152 -7.37342014009519e-11 0 0;-0.00148 -7.20026891471466e-11 0 0;-0.00144 -7.02548041027539e-11 0 0;-0.0014 -6.849094372176e-11 0 0;-0.00136 -6.67115090908044e-11 0 0;-0.00132 -6.49169048379772e-11 0 0;-0.00128 -6.31075390408094e-11 0 0;-0.00124 -6.12838231334798e-11 0 0;-0.0012 -5.9446171813259e-11 0 0;-0.00116 -5.75950029462097e-11 0 0;-0.00112 -5.57307374721687e-11 0 0;-0.00108 -5.38537993090279e-11 0 0;-0.00104 -5.19646152563396e-11 0 0;-0.001 -5.00636148982657e-11 4695.72941749421 -13362.2957077408;-0.00096 -4.81512305058942e-11 4896.68712230303 -13289.9688778721;-0.00092 -4.62278969389442e-11 5096.53136268747 -13214.6200236884;-0.00088 -4.42940515468827e-11 5295.21669579065 -13136.2662788693;-0.00084 -4.23501340694751e-11 5492.69794228121 -13054.9254603807;-0.0008 -4.0396586536792e-11 5688.93019662671 -12970.6160644233;-0.00076 -3.84338531686959e-11 5883.86883730474 -12883.3572622267;-0.00072 -3.64623802738286e-11 6077.46953694948 -12793.1688956901;-0.00068 -3.44826161481252e-11 6269.68827243139 -12700.0714728701;-0.00064 -3.24950109728751e-11 6460.48133486764 -12604.0861633179;-0.0006 -3.05000167123548e-11 6649.80533956116 -12505.2347932652;-0.00056 -2.84980870110551e-11 6837.61723586594 -12403.5398406611;-0.00052 -2.64896770905262e-11 7023.87431697638 -12299.0244300608;-0.00048 -2.4475243645864e-11 7208.53422963846 -12191.7123273674;-0.00044 -2.24552447418623e-11 7391.55498378047 -12081.6279344275;-0.0004 -2.04301397088522e-11 7572.89496206122 -11968.7962834829;-0.00036 -1.84003890382542e-11 7752.51292933346 -11853.243031478;-0.00032 -1.63664542778671e-11 7930.3680420204 -11734.9944542257;-0.00028 -1.43287979269155e-11 8106.41985740317 -11614.0774404328;-0.00024 -1.22878833308817e-11 8280.62834281714 -11490.5194855854;-0.0002 -1.02441745761446e-11 8452.95388475506 -11364.3486856971;-0.00016 -8.19813638445086e-12 8623.35729787476 -11235.5937309196;-0.00012 -6.15023400724103e-12 8791.79983390958 -11104.2838990193;-8e-05 -4.10093311985532e-12 8958.24319047943 -10970.4490487197;-4e-05 -2.05069971564309e-12 9122.64951980036 -10834.1196129115]  x5=0.00157786097191812  V1=ones(3,3)  V2=ones(3,3)  I1=ones(3,3)  I2=ones(3,3)  nHarmo=1  Measurements=None  Decoupling=off  VsMag0=0  VrMag0=0  VsAngle0=0  VrAngle0=0  IsMag0=0  IrMag0=0  IsAngle0=0  IrAngle0=0
      settings: AttributesFormatString=\n
  LG2_5500 MVA : powerlib/Machines/Synchronous Machine pu Standard  PresetModel=No  MechanicalLoad=Mechanical power Pm  ShowDetailedParameters=on  RotorType=Salient-pole  Units=per unit standard parameters  MeasurementBus=off  NominalParameters="[5500E6  13800   60 ]"  Reactances1=[ 31 32 33 34 35 36 37 ]  Reactances2=[ 1.305, 0.296, 0.252, 0.474, 0.243, 0.18 ]  dAxisTimeConstants=Short-circuit  qAxisTimeConstants=Open-circuit  TimeConstants1=[]  TimeConstants2=[]  TimeConstants3=[]  TimeConstants4=[]  TimeConstants5=[ 1.01, 0.053, 0.1 ]  TimeConstants6=[]  TimeConstants7=[]  TimeConstants8=[]  StatorResistance=2.8544e-3  Mechanical="[ 4.1  0  32]"  PolePairs=32  InitialConditions=[0 -68.2322 0.822292 0.822292 0.822292 4.1842 -115.816 124.184 1.25511]  SetSaturation=off  Saturation=[0.6404,0.7127,0.8441,0.9214,0.9956,1.082,1.19,1.316,1.457;0.7,0.7698,0.8872,0.9466,0.9969,1.046,1.1,1.151,1.201]  LoadFlowParameters=[2 4000000000 0 0 0]  TsPowergui=0  TsBlock=-1  IterativeModel=Trapezoidal non iterative  IterativeDiscreteModel=Trapezoidal non iterative  BusType=swing  Pref=0  Qref=0  Qmin=-Inf  Qmax=Inf  PLF=0  QLF=0
      settings: AttributesFormatString=\n\n
  LG3 660 Mvar : powerlib/Elements/Three-Phase Series RLC Load  LConnTagsString=A|B|C  Configuration=Y (grounded)  NominalVoltage=735e3  Vabc=[1e3 1e3 1e3]  Vabcp=[1e3 1e3 1e3]  NominalFrequency=60  UnbalancedPower=off  ActivePower=2200000  InductivePower=660e6  CapacitivePower=0  Pabc=[10e3 9e3 11e3]  QLabc=[100 90 110]  QCabc=[100 90 110]  Pabcp=[10e3 9e3 11e3]  QLabcp=[100 90 110]  QCabcp=[100 90 110]  Measurements=None  LoadType=constant Z
  LG3-LMO 104km : powerlib/Elements/Distributed Parameters Line  Phases=3  Length=104  Frequency=60  Resistance="[0.01273  0.3864]"  Inductance="[0.9337e-3  4.1264e-3]"  Capacitance=[12.74e-9 7.751e-9]  x1=[-0.0006 -1.84830263941326e-09 0 0;-0.00056 -1.86396339240874e-09 0 0;-0.00052 -1.87920029620293e-09 0 0;-0.00048 -1.89400988605529e-09 0 0;-0.00044 -1.90838879439281e-09 0 0;-0.0004 -1.92233375157573e-09 0 0;-0.00036 -1.93584158664104e-09 550361.292729844 -486648.874020019;-0.00032 -1.94890922802354e-09 557636.96604459 -478294.603153812;-0.00028 -1.96153370425426e-09 564785.837522115 -469831.572219484;-0.00024 -1.97371214463618e-09 571806.281570693 -461261.705637289;-0.0002 -1.98544177989698e-09 578696.701801889 -452586.952120983;-0.00016 -1.99671994281875e-09 585455.531393563 -443809.284234708;-0.00012 -2.0075440688445e-09 592081.233446151 -434930.697944447;-8e-05 -2.01791169666132e-09 598572.301332146 -425953.212164156;-4e-05 -2.02782046876005e-09 604927.259038684 -416878.868296683]  x2=[-0.0006 -1.03652618900468e-08 0 0;-0.00056 -1.03424105982859e-08 0 0;-0.00052 -1.03172075315441e-08 0 0;-0.00048 -1.02896584207814e-08 0 0;-0.00044 -1.0259769530428e-08 0 0;-0.0004 -1.022754765696e-08 0 0;-0.00036 -1.01930001273533e-08 509416.858098534 -556033.052302243;-0.00032 -1.01561347974184e-08 517743.436837333 -548288.300411814;-0.00028 -1.01169600500133e-08 525952.285183424 -540418.872490108;-0.00024 -1.00754847931378e-08 534041.536515484 -532426.557977173;-0.0002 -1.00317184579076e-08 542009.351407518 -524313.174256404;-0.00016 -9.98567099640994e-09 549853.918047132 -516080.566241293;-0.00012 -9.93735287944046e-09 557573.45264752 -507730.605955909;-8e-05 -9.88677509412227e-09 565166.199853084 -499265.192109212;-4e-05 -9.83394914140759e-09 572630.433138588 -490686.249663309]  x3=[-0.0006 -2.5891516730553e-11 0 0;-0.00056 -2.65642269247652e-11 0 0;-0.00052 -2.72308966428549e-11 0 0;-0.00048 -2.78913742898772e-11 0 0;-0.00044 -2.8545509678911e-11 0 0;-0.0004 -2.91931540652098e-11 0 0;-0.00036 -2.98341601800252e-11 -30.215477134681 -878.894027383642;-0.00032 -3.04683822640945e-11 -16.958916126324 -879.249677062614;-0.00028 -3.10956761007851e-11 -3.69849880668731 -879.405392947349;-0.00024 -3.1715899048888e-11 9.5627595196835 -879.361139629396;-0.0002 -3.23289100750535e-11 22.8218433570053 -879.116927171579;-0.00016 -3.29345697858606e-11 36.0757377039548 -878.672811105705;-0.00012 -3.3532740459514e-11 49.3214287392544 -878.028892419937;-8e-05 -3.4123286077161e-11 62.5559045069886 -877.185317535831;-4e-05 -3.47060723538207e-11 75.7761556014971 -876.142278275042]  x4=[-0.0006 1.25600763098792e-11 0 0;-0.00056 1.32080406000832e-11 0 0;-0.00052 1.3853001495756e-11 0 0;-0.00048 1.44948123383518e-11 0 0;-0.00044 1.51333271856198e-11 0 0;-0.0004 1.57684008447901e-11 0 0;-0.00036 1.63998889055892e-11 3670.37159989901 -3222.94831504442;-0.00032 1.70276477730778e-11 3718.55339649164 -3167.23609882145;-0.00028 1.76515347003029e-11 3765.88962610934 -3110.80368042269;-0.00024 1.82714078207575e-11 3812.36952490171 -3053.66389209344;-0.0002 1.88871261806397e-11 3857.98252374059 -2995.82972692879;-0.00016 1.94985497709039e-11 3902.7182506234 -2937.31433591918;-0.00012 2.01055395590986e-11 3946.56653303163 -2878.13102495989;-8e-05 2.07079575209804e-11 3989.51740024398 -2818.29325182548;-4e-05 2.13056666718997e-11 4031.56108560365 -2757.81462310953]  x5=0.000588163229675572  V1=ones(3,3)  V2=ones(3,3)  I1=ones(3,3)  I2=ones(3,3)  nHarmo=1  Measurements=None  Decoupling=off  VsMag0=0  VrMag0=0  VsAngle0=0  VrAngle0=0  IsMag0=0  IrMag0=0  IsAngle0=0  IrAngle0=0
      settings: AttributesFormatString=\n
  LG31-200 MVA : powerlib/Machines/Synchronous Machine pu Standard  PresetModel=No  MechanicalLoad=Mechanical power Pm  ShowDetailedParameters=on  RotorType=Salient-pole  Units=per unit standard parameters  MeasurementBus=off  NominalParameters="[200E6  13800   60 ]"  Reactances1=[ 31 32 33 34 35 36 37 ]  Reactances2=[ 1.305, 0.296, 0.252, 0.474, 0.243, 0.18 ]  dAxisTimeConstants=Short-circuit  qAxisTimeConstants=Open-circuit  TimeConstants1=[]  TimeConstants2=[]  TimeConstants3=[]  TimeConstants4=[]  TimeConstants5=[ 1.01, 0.053, 0.1 ]  TimeConstants6=[]  TimeConstants7=[]  TimeConstants8=[]  StatorResistance=2.8544e-3  Mechanical="[ 3.2  0  32]"  PolePairs=32  InitialConditions=[0 -65.0253 0.900243 0.900243 0.900243 0.798134 -119.202 120.798 1.40505]  SetSaturation=off  Saturation=[0.6404,0.7127,0.8441,0.9214,0.9956,1.082,1.19,1.316,1.457;0.7,0.7698,0.8872,0.9466,0.9969,1.046,1.1,1.151,1.201]  LoadFlowParameters=[1 180000000 0 0 0]  TsPowergui=0  TsBlock=-1  IterativeModel=Trapezoidal non iterative  IterativeDiscreteModel=Trapezoidal non iterative  BusType=PV  Pref=180000000  Qref=0  Qmin=-Inf  Qmax=Inf  PLF=0  QLF=0
      settings: AttributesFormatString=\n\n
  LG3_2200 MVA : powerlib/Machines/Synchronous Machine pu Standard  PresetModel=No  MechanicalLoad=Mechanical power Pm  ShowDetailedParameters=on  RotorType=Salient-pole  Units=per unit standard parameters  MeasurementBus=off  NominalParameters="[2200E6  13800   60 ]"  Reactances1=[ 31 32 33 34 35 36 37 ]  Reactances2=[ 1.305, 0.296, 0.252, 0.474, 0.243, 0.18 ]  dAxisTimeConstants=Short-circuit  qAxisTimeConstants=Open-circuit  TimeConstants1=[]  TimeConstants2=[]  TimeConstants3=[]  TimeConstants4=[]  TimeConstants5=[ 1.01, 0.053, 0.1 ]  TimeConstants6=[]  TimeConstants7=[]  TimeConstants8=[]  StatorResistance=2.8544e-3  Mechanical="[ 3.2  0  32]"  PolePairs=32  InitialConditions=[0 -67.4267 0.818333 0.818333 0.818333 0.465769 -119.534 120.466 1.33761]  SetSaturation=off  Saturation=[0.6404,0.7127,0.8441,0.9214,0.9956,1.082,1.19,1.316,1.457;0.7,0.7698,0.8872,0.9466,0.9969,1.046,1.1,1.151,1.201]  LoadFlowParameters=[1 1800000000 0 0 0]  TsPowergui=0  TsBlock=-1  IterativeModel=Trapezoidal non iterative  IterativeDiscreteModel=Trapezoidal non iterative  BusType=PV  Pref=1800000000  Qref=0  Qmin=-Inf  Qmax=Inf  PLF=0  QLF=0
      settings: AttributesFormatString=\n\n
  LG4 660 Mvar : powerlib/Elements/Three-Phase Series RLC Load  LConnTagsString=A|B|C  Configuration=Y (grounded)  NominalVoltage=735e3  Vabc=[1e3 1e3 1e3]  Vabcp=[1e3 1e3 1e3]  NominalFrequency=60  UnbalancedPower=off  ActivePower=2200000  InductivePower=660e6  CapacitivePower=0  Pabc=[10e3 9e3 11e3]  QLabc=[100 90 110]  QCabc=[100 90 110]  Pabcp=[10e3 9e3 11e3]  QLabcp=[100 90 110]  QCabcp=[100 90 110]  Measurements=None  LoadType=constant Z
  LG4-2700 MVA : powerlib/Machines/Synchronous Machine pu Standard  PresetModel=No  MechanicalLoad=Mechanical power Pm  ShowDetailedParameters=on  RotorType=Salient-pole  Units=per unit standard parameters  MeasurementBus=off  NominalParameters="[2700E6  13800   60 ]"  Reactances1=[ 31 32 33 34 35 36 37 ]  Reactances2=[ 1.305, 0.296, 0.252, 0.474, 0.243, 0.18 ]  dAxisTimeConstants=Short-circuit  qAxisTimeConstants=Open-circuit  TimeConstants1=[]  TimeConstants2=[]  TimeConstants3=[]  TimeConstants4=[]  TimeConstants5=[ 1.01, 0.053, 0.1 ]  TimeConstants6=[]  TimeConstants7=[]  TimeConstants8=[]  StatorResistance=2.8544e-3  Mechanical="[ 3.7  0  32]"  PolePairs=32  InitialConditions=[0 -66.0751 0.928325 0.928325 0.928325 3.71347 -116.287 123.713 1.33221]  SetSaturation=off  Saturation=[0.6404,0.7127,0.8441,0.9214,0.9956,1.082,1.19,1.316,1.457;0.7,0.7698,0.8872,0.9466,0.9969,1.046,1.1,1.151,1.201]  LoadFlowParameters=[1 2500000000 0 0 0]  TsPowergui=0  TsBlock=-1  IterativeModel=Trapezoidal non iterative  IterativeDiscreteModel=Trapezoidal non iterative  BusType=PV  Pref=2500000000  Qref=0  Qmin=-Inf  Qmax=Inf  PLF=0  QLF=0
      settings: AttributesFormatString=\n\n
  LG4-LMO 3*118km : powerlib/Elements/Distributed Parameters Line  Phases=3  Length=118  Frequency=60  Resistance="[0.01273  0.3864]/3"  Inductance="[0.9337e-3  4.1264e-3]/3"  Capacitance=[12.74e-9 7.751e-9]*3  x1=[-0.00068 -4.18210065310314e-09 0 0;-0.00064 -4.17989429564359e-09 0 0;-0.0006 -4.17673746626708e-09 0 0;-0.00056 -4.1726308828094e-09 0 0;-0.00052 -4.1675754790722e-09 0 0;-0.00048 -4.1615724046107e-09 0 0;-0.00044 -4.15462302447226e-09 516886.507539444 -533088.832051592;-0.0004 -4.14672891888601e-09 524866.260234349 -525234.058895319;-0.00036 -4.13789188290346e-09 532726.662867931 -517259.852043478;-0.00032 -4.1281139259904e-09 540465.928052416 -509168.024761942;-0.00028 -4.11739727156991e-09 548082.295945641 -500960.417062454;-0.00024 -4.10574435651679e-09 555574.034651229 -492638.895284224;-0.0002 -4.09315783060342e-09 562939.440612403 -484205.351669543;-0.00016 -4.07964055589727e-09 570176.838999365 -475661.703933501;-0.00012 -4.06519560611002e-09 577284.584090135 -467009.894827917;-8e-05 -4.04982626589871e-09 584261.059644772 -458251.891699571;-4e-05 -4.03353603011874e-09 591104.679272899 -449389.686042849]  x2=[-0.00068 -1.01947908065967e-08 0 0;-0.00064 -1.01731333123589e-08 0 0;-0.0006 -1.01491625353353e-08 0 0;-0.00056 -1.01228839262737e-08 0 0;-0.00052 -1.00943034607034e-08 0 0;-0.00048 -1.00634276375757e-08 0 0;-0.00044 -1.00302634777865e-08 492418.109351948 -571141.512380813;-0.0004 -9.99481852257972e-09 500974.442359227 -563651.367071603;-0.00036 -9.95710083183257e-09 509416.858098534 -556033.052302243;-0.00032 -9.91711898222265e-09 517743.436837332 -548288.300411814;-0.00028 -9.87488206527776e-09 525952.285183423 -540418.872490108;-0.00024 -9.83039968530859e-09 534041.536515483 -532426.557977173;-0.0002 -9.78368195722472e-09 542009.351407518 -524313.174256404;-0.00016 -9.73473950423467e-09 549853.918047131 -516080.566241293;-0.00012 -9.68358345543018e-09 557573.452647519 -507730.605955909;-8e-05 -9.63022544325558e-09 565166.199853084 -499265.192109212;-4e-05 -9.57467760086272e-09 572630.433138588 -490686.249663309]  x3=[-0.00068 -5.67102090860295e-11 0 0;-0.00064 -5.80547125775572e-11 0 0;-0.0006 -5.93860149280872e-11 0 0;-0.00056 -6.07038134109459e-11 0 0;-0.00052 -6.20078083701222e-11 0 0;-0.00048 -6.32977032884078e-11 0 0;-0.00044 -6.45732048548217e-11 2439.66221449871 -4653.8550715936;-0.0004 -6.58340230313072e-11 2509.56057642805 -4616.53818276402;-0.00036 -6.70798711186839e-11 2578.88828592383 -4578.17153296301;-0.00032 -6.83104658218403e-11 2647.62957846278 -4538.76384643587;-0.00028 -6.95255273141532e-11 2715.76882286778 -4498.32408415068;-0.00024 -7.07247793011175e-11 2783.29052486225 -4456.86144176066;-0.0002 -7.19079490831733e-11 2850.17933059343 -4414.38534751311;-0.00016 -7.30747676177152e-11 2916.42003012374 -4370.90546010558;-0.00012 -7.42249695802709e-11 2981.99756088934 -4326.4316664895;-8e-05 -7.53582934248329e-11 3046.89701112524 -4280.97407962202;-4e-05 -7.64744814433323e-11 3111.10362325614 -4234.54303616638]  x4=[-0.00068 4.28549778379221e-12 0 0;-0.00064 5.68983883964163e-12 0 0;-0.0006 7.09288607520599e-12 0 0;-0.00056 8.4943204496433e-12 0 0;-0.00052 9.89382328886225e-12 0 0;-0.00048 1.1291076357986e-11 0 0;-0.00044 1.26857619337161e-11 7760.55546915048 -8389.19553240714;-0.0004 1.40775628765798e-11 7886.17526885014 -8271.21966069501;-0.00036 1.5466162703045e-11 8010.00182030114 -8151.36298495999;-0.00032 1.68512456574862e-11 8132.00696641352 -8029.65275957655;-0.00028 1.82324967839837e-11 8252.16296426917 -7906.11666040037;-0.00024 1.96096019979429e-11 8370.44249143038 -7780.78277847505;-0.0002 2.09822481575139e-11 8486.81865215265 -7653.67961364452;-0.00016 2.23501231347969e-11 8601.26498350063 -7524.83606807237;-0.00012 2.37129158868184e-11 8713.75546136552 -7394.28143966977;-8e-05 2.50703165262587e-11 8824.26450638272 -7262.04541543335;-4e-05 2.64220163919182e-11 8932.76698974838 -7128.15806469467]  x5=0.000667339049054976  V1=ones(3,3)  V2=ones(3,3)  I1=ones(3,3)  I2=ones(3,3)  nHarmo=1  Measurements=None  Decoupling=off  VsMag0=0  VrMag0=0  VsAngle0=0  VrAngle0=0  IsMag0=0  IrMag0=0  IsAngle0=0  IrAngle0=0
      settings: AttributesFormatString=\n
  LMO 330 Mvar : powerlib/Elements/Three-Phase Series RLC Load  LConnTagsString=A|B|C  Configuration=Y (grounded)  NominalVoltage=735e3  Vabc=[1e3 1e3 1e3]  Vabcp=[1e3 1e3 1e3]  NominalFrequency=60  UnbalancedPower=off  ActivePower=1100000  InductivePower=330e6  CapacitivePower=0  Pabc=[10e3 9e3 11e3]  QLabc=[100 90 110]  QCabc=[100 90 110]  Pabcp=[10e3 9e3 11e3]  QLabcp=[100 90 110]  QCabcp=[100 90 110]  Measurements=None  LoadType=constant Z
  LMO-ALB 3*218km : powerlib/Elements/Distributed Parameters Line  Phases=3  Length=218  Frequency=60  Resistance="[0.01273  0.3864]/3"  Inductance="[0.9337e-3  4.1264e-3]/3"  Capacitance=[12.74e-9 7.751e-9]*3  x1=[-0.00124 -1.02694510590558e-08 300539.143349663 -691631.439094573;-0.0012 -1.02809455251556e-08 310934.166982951 -687020.941454274;-0.00116 -1.02901021929021e-08 321258.48686805 -682254.221176505;-0.00112 -1.0296918980148e-08 331509.755343649 -677332.36217235;-0.00108 -1.03013943368147e-08 341685.641359702 -672256.483630103;-0.00104 -1.03035272452446e-08 351783.831007481 -667027.739760771;-0.001 -1.03033172204328e-08 361802.028045744 -661647.31953562;-0.00096 -1.03007643101371e-08 371737.954422877 -656116.44641581;-0.00092 -1.02958690948672e-08 381589.350794905 -650436.378074192;-0.00088 -1.0288632687753e-08 391353.977039249 -644608.406109325;-0.00084 -1.0279056734291e-08 401029.612764108 -638633.855751774;-0.0008 -1.02671434119704e-08 410614.057813356 -632514.08556277;-0.00076 -1.0252895429778e-08 420105.132766842 -626250.487125277;-0.00072 -1.02363160275821e-08 429500.679435969 -619844.484727567;-0.00068 -1.02174089753958e-08 438798.561354449 -613297.53503934;-0.00064 -1.01961785725196e-08 447996.664264114 -606611.126780499;-0.0006 -1.01726296465641e-08 457092.896595685 -599786.780382619;-0.00056 -1.0146767552352e-08 466085.189944371 -592826.047643221;-0.00052 -1.01185981707005e-08 474971.49954021 -585730.511372902;-0.00048 -1.00881279070841e-08 483749.804713035 -578501.785035423;-0.00044 -1.00553636901779e-08 492418.109351948 -571141.512380813;-0.0004 -1.00203129702823e-08 500974.442359227 -563651.367071603;-0.00036 -9.98298371762877e-09 509416.858098534 -556033.052302243;-0.00032 -9.94338442056745e-09 517743.436837332 -548288.300411814;-0.00028 -9.90152408363698e-09 525952.285183423 -540418.872490108;-0.00024 -9.857412225517e-09 534041.536515483 -532426.557977173;-0.0002 -9.81105887686363e-09 542009.351407518 -524313.174256404;-0.00016 -9.76247457802864e-09 549853.918047131 -516080.566241293;-0.00012 -9.7116703766626e-09 557573.452647519 -507730.605955909;-8e-05 -9.65865782520279e-09 565166.199853084 -499265.192109212;-4e-05 -9.60344897824624e-09 572630.433138588 -490686.249663309]  x2=[-0.00124 -2.61572435918466e-08 180359.157644875 -744264.312743924;-0.0012 -2.61714780920089e-08 191561.495110717 -741460.025520107;-0.00116 -2.61797614237463e-08 202720.273144527 -738487.136680566;-0.00112 -2.61820917035005e-08 213832.954336409 -735346.322234586;-0.00108 -2.61784684013861e-08 224897.011758492 -732038.296376286;-0.00104 -2.61688923413108e-08 235909.92953953 -728563.811322219;-0.001 -2.61533657007879e-08 246869.203436992 -724923.657140325;-0.00096 -2.61318920104417e-08 257772.341406501 -721118.661570272;-0.00092 -2.61044761532042e-08 268616.864168509 -717149.689835241;-0.00088 -2.60711243632048e-08 279400.305772057 -713017.644445177;-0.00084 -2.6031844224353e-08 290120.214155519 -708723.464991568;-0.0008 -2.59866446686137e-08 300774.151704172 -704268.127933791;-0.00076 -2.59355359739761e-08 311359.695804493 -699652.646377071;-0.00072 -2.58785297621165e-08 321874.43939504 -694878.069842113;-0.00068 -2.58156389957559e-08 332315.991513796 -689945.484026446;-0.00064 -2.57468779757122e-08 342681.977841852 -684856.010557548;-0.0006 -2.56722623376485e-08 352970.04124331 -679610.806737795;-0.00056 -2.55918090485174e-08 363177.842301274 -674211.065281305;-0.00052 -2.55055364027031e-08 373303.059849811 -668658.014042718;-0.00048 -2.54134640178611e-08 383343.391501767 -662952.915737999;-0.00044 -2.53156128304578e-08 393296.554172307 -657097.067657304;-0.0004 -2.52120050910095e-08 403160.284598074 -651091.801369987;-0.00036 -2.51026643590225e-08 412932.33985183 -644938.482421815;-0.00032 -2.49876154976364e-08 422610.49785248 -638638.510024453;-0.00028 -2.48668846679702e-08 432192.557870356 -632193.316737295;-0.00024 -2.47404993231734e-08 441676.341027642 -625604.368141714;-0.0002 -2.46084882021835e-08 451059.690793833 -618873.162507801;-0.00016 -2.44708813231909e-08 460340.473476111 -612001.230453667;-0.00012 -2.43277099768134e-08 469516.578704527 -604990.134597403;-8e-05 -2.41790067189803e-08 478585.919911885 -597841.469201743;-4e-05 -2.40248053635303e-08 487546.434808203 -590556.859811553]  x3=[-0.00124 -6.51078489767314e-11 -23.6154950485161 -3420.19245712882;-0.0012 -6.72418516337065e-11 27.9605314525414 -3420.159718588;-0.00116 -6.9360564073489e-11 79.5301999698679 -3419.34926522137;-0.00112 -7.14635045191413e-11 131.081784005561 -3417.76128131905;-0.00108 -7.35501947801409e-11 182.603561173971 -3415.39612797487;-0.00104 -7.56201603611174e-11 234.083815867277 -3412.25434300431;-0.001 -7.76729305697482e-11 285.510841919508 -3408.33664082218;-0.00096 -7.97080386237903e-11 336.872945268426 -3403.64391228017;-0.00092 -8.17250217572223e-11 388.158446614659 -3398.17722446428;-0.00088 -8.37234213254732e-11 439.355684077468 -3391.93782045218;-0.00084 -8.57027829097147e-11 490.45301584656 -3384.92711903053;-0.0008 -8.76626564201918e-11 541.438822829335 -3377.14671437239;-0.00076 -8.96025961985696e-11 592.301511292968 -3368.59837567467;-0.00072 -9.15221611192717e-11 643.029515500724 -3359.28404675588;-0.00068 -9.34209146897888e-11 693.611300341905 -3349.20584561409;-0.00064 -9.52984251499331e-11 744.035363954837 -3338.36606394532;-0.0006 -9.71542655700169e-11 794.290240342295 -3326.76716662246;-0.00056 -9.89880139479328e-11 844.364501978765 -3314.41179113473;-0.00052 -1.00799253305113e-10 894.246762408975 -3301.30274698796;-0.00048 -1.02587571781348e-10 943.925678837068 -3287.44301506575;-0.00044 -1.04352562728437e-10 993.389954705863 -3272.83574695161;-0.0004 -1.06093824802659e-10 1042.62834226559 -3257.48426421235;-0.00036 -1.07810962056036e-10 1091.62964513152 -3241.39205764276;-0.00032 -1.09503584026364e-10 1140.38272082997 -3224.56278647183;-0.00028 -1.11171305826002e-10 1188.87648333194 -3207.00027753071;-0.00024 -1.12813748229396e-10 1237.09990557404 -3188.70852438247;-0.0002 -1.14430537759307e-10 1285.04202196591 -3169.69168641403;-0.00016 -1.16021306771739e-10 1332.69193088371 -3149.95408789036;-0.00012 -1.17585693539536e-10 1380.03879714907 -3129.50021697115;-8e-05 -1.19123342334638e-10 1427.07185449291 -3108.33472469026;-4e-05 -1.20633903508969e-10 1473.78040800358 -3086.46242389812]  x4=[-0.00124 -6.81469550440532e-11 3052.91388647933 -13125.6647014601;-0.0012 -6.66205804503875e-11 3250.49024737168 -13078.1368217797;-0.00116 -6.50790569112388e-11 3447.3274748128 -13027.6350865671;-0.00112 -6.35227349557664e-11 3643.38080971464 -12974.1709794814;-0.00108 -6.19519684781617e-11 3838.60567123953 -12917.7566577994;-0.00104 -6.03671146571762e-11 4032.95766693751 -12858.4049496514;-0.001 -5.87685338749014e-11 4226.39260284076 -12796.1293511041;-0.00096 -5.71565896348217e-11 4418.86649351299 -12730.9440230914;-0.00092 -5.55316484791565e-11 4610.33557205128 -12662.8637881948;-0.00088 -5.38940799055117e-11 4800.75630003832 -12591.9041272727;-0.00084 -5.22442562828591e-11 4990.0853774427 -12518.08117594;-0.0008 -5.05825527668631e-11 5178.2797524649 -12441.4117208992;-0.00076 -4.89093472145732e-11 5365.29663132698 -12361.9131961233;-0.00072 -4.7225020098503e-11 5551.09348800344 -12279.6036788911;-0.00068 -4.55299544201136e-11 5735.62807389132 -12194.5018856772;-0.00064 -4.38245356227227e-11 5918.85842741715 -12106.6271678954;-0.0006 -4.21091515038579e-11 6100.74288357865 -12015.9995074987;-0.00056 -4.0384192127075e-11 6281.24008341898 -11922.6395124356;-0.00052 -3.86500497332608e-11 6460.30898343146 -11826.5684119638;-0.00048 -3.69071186514411e-11 6637.90886489243 -11727.8080518231;-0.00044 -3.51557952091135e-11 6813.99934312042 -11626.3808892677;-0.0004 -3.3396477642126e-11 6988.5403766592 -11522.3099879597;-0.00036 -3.16295660041217e-11 7161.49227638294 -11415.6190127247;-0.00032 -2.98554620755697e-11 7332.81571452111 -11306.3322241703;-0.00028 -2.80745692724044e-11 7502.47173360131 -11194.4744731697;-0.00024 -2.62872925542912e-11 7670.42175530784 -11080.071195211;-0.0002 -2.44940383325432e-11 7836.62758925412 -10963.148404613;-0.00016 -2.26952143777059e-11 8001.05144166681 -10843.7326886099;-0.00012 -2.08912297268344e-11 8163.65592397978 -10721.8512013058;-8e-05 -1.90824945904812e-11 8324.40406133601 -10597.5316574998;-4e-05 -1.72694202594186e-11 8483.2593009953 -10470.8023263841]  x5=0.00123288061605072  V1=ones(3,3)  V2=ones(3,3)  I1=ones(3,3)  I2=ones(3,3)  nHarmo=1  Measurements=None  Decoupling=off  VsMag0=0  VrMag0=0  VsAngle0=0  VrAngle0=0  IsMag0=0  IrMag0=0  IsAngle0=0  IrAngle0=0
      settings: AttributesFormatString=\n
  LMO7 : powerlib/Measurements/Three-Phase V-I Measurement  VoltageMeasurement=no  SetLabelV=on  LabelV=Vabc_LMO7  Vpu=on  VpuLL=off  CurrentMeasurement=no  SetLabelI=off  LabelI=A1  Ipu=off  Pbase=100e6  Vbase=735e3  OutputType=Magnitude  PhasorSimulation=off  PSBequivalent=0
  LVD 990 Mvar : powerlib/Elements/Three-Phase Series RLC Load  LConnTagsString=A|B|C  Configuration=Y (grounded)  NominalVoltage=735e3  Vabc=[1e3 1e3 1e3]  Vabcp=[1e3 1e3 1e3]  NominalFrequency=60  UnbalancedPower=off  ActivePower=3300000  InductivePower=990e6  CapacitivePower=0  Pabc=[10e3 9e3 11e3]  QLabc=[100 90 110]  QCabc=[100 90 110]  Pabcp=[10e3 9e3 11e3]  QLabcp=[100 90 110]  QCabcp=[100 90 110]  Measurements=None  LoadType=constant Z
  LVD-MTL 3*260km : powerlib/Elements/Distributed Parameters Line  Phases=3  Length=260  Frequency=60  Resistance="[0.01273  0.3864]/3"  Inductance="[0.9337e-3  4.1264e-3]/3"  Capacitance=[12.74e-9 7.751e-9]*3  x1=[-0.00148 -8.42989571824446e-08 -29973.8950595762 -777968.644211176;-0.00144 -8.44624312099071e-08 -18239.4210690995 -778332.14588106;-0.0014 -8.46066992088854e-08 -6500.79959156173 -778518.66153302;-0.00136 -8.47317283740808e-08 5239.30011174263 -778528.148755008;-0.00132 -8.48374902749391e-08 16978.2084433834 -778360.605389709;-0.00128 -8.49239608621163e-08 28713.2560768381 -778016.069535041;-0.00124 -8.49911204729465e-08 40441.7745634733 -777494.619535485;-0.0012 -8.50389538359134e-08 52161.0969393279 -776796.373964275;-0.00116 -8.50674500741227e-08 63868.5583315566 -775921.491596431;-0.00112 -8.50766027077755e-08 75561.4965643996 -774870.171372661;-0.00108 -8.5066409655642e-08 87237.2527645385 -773642.652354117;-0.00104 -8.50368732355343e-08 98893.1719657009 -772239.213668037;-0.001 -8.49880001637796e-08 110526.603712377 -770660.174444277;-0.00096 -8.49198015536929e-08 122134.902662509 -768905.893742738;-0.00092 -8.48322929130501e-08 133715.429189022 -766976.770471724;-0.00088 -8.47254941405614e-08 145265.549980051 -764873.243297231;-0.00084 -8.45994295213467e-08 156782.638637731 -762595.790543198;-0.0008 -8.44541277214132e-08 168264.07627542 -760144.930082741;-0.00076 -8.42896217811373e-08 179707.252113213 -757521.219220394;-0.00072 -8.41059491077511e-08 191109.564071603 -754725.254565382;-0.00068 -8.39031514668366e-08 202468.419363183 -751757.671895954;-0.00064 -8.36812749728285e-08 213781.235082213 -748619.14601482;-0.0006 -8.34403700785282e-08 225045.438791956 -745310.390595698;-0.00056 -8.31804915636311e-08 236258.469109627 -741832.158021038;-0.00052 -8.29016985222704e-08 247417.776288829 -738185.239210932;-0.00048 -8.26040543495796e-08 258520.822799342 -734370.463443268;-0.00044 -8.22876267272767e-08 269565.08390414 -730388.698165158;-0.0004 -8.19524876082743e-08 280548.048233488 -726240.848795689;-0.00036 -8.15987132003179e-08 291467.218356011 -721927.858520038;-0.00032 -8.12263839486571e-08 302320.111346586 -717450.708075;-0.00028 -8.08355845177529e-08 313104.259350939 -712810.415525978;-0.00024 -8.04264037720257e-08 323817.210146811 -708008.03603548;-0.0002 -7.99989347556486e-08 334456.527701577 -703044.661623189;-0.00016 -7.95532746713895e-08 345019.792726173 -697921.420917644;-0.00012 -7.90895248585083e-08 355504.603225228 -692639.4788996;-8e-05 -7.86077907697132e-08 365908.57504325 -687200.036637123;-4e-05 -7.81081819471819e-08 376229.342406769 -681604.331012476]  x2=[-0.00148 -1.25190246548987e-07 -239041.03098161 -695044.447394225;-0.00144 -1.25375650094684e-07 -228533.218022323 -698569.915440381;-0.0014 -1.25532544298743e-07 -217973.438580045 -701936.534711976;-0.00136 -1.25660893484775e-07 -207364.093857557 -705143.539668821;-0.00132 -1.25760668467282e-07 -196707.596328357 -708190.201065644;-0.00128 -1.25831846558293e-07 -186006.369188086 -711075.826117917;-0.00124 -1.25874411572525e-07 -175262.845803513 -713799.758659387;-0.0012 -1.2588835383106e-07 -164479.469159206 -716361.379291285;-0.00116 -1.25873670163548e-07 -153658.691302023 -718760.10552317;-0.00112 -1.2583036390893e-07 -142802.972783534 -720995.391905382;-0.00108 -1.25758444914673e-07 -131914.782100515 -723066.730153074;-0.00104 -1.25657929534538e-07 -120996.59513363 -724973.649261791;-0.001 -1.25528840624854e-07 -110050.894584442 -726715.715614573;-0.00096 -1.25371207539327e-07 -99080.1694108642 -728292.533080553;-0.00092 -1.25185066122361e-07 -88086.9142611933 -729703.743105039;-0.00088 -1.24970458700908e-07 -77073.6289068486 -730949.024791039;-0.00084 -1.24727434074846e-07 -66042.8176739452 -732028.094972237;-0.0008 -1.2445604750588e-07 -54996.9888738317 -732940.70827738;-0.00076 -1.24156360704973e-07 -43938.6542327221 -733686.657186073;-0.00072 -1.23828441818321e-07 -32870.3283205508 -734265.772075965;-0.00068 -1.23472365411851e-07 -21794.5279791811 -734677.921261326;-0.00064 -1.23088212454266e-07 -10713.7717500969 -734923.011022985;-0.0006 -1.22676070298637e-07 369.420698291617 -735000.985629643;-0.00056 -1.22236032662535e-07 11452.5291435991 -734911.827350547;-0.00052 -1.21768199606724e-07 22533.0333825417 -734655.556459522;-0.00048 -1.21272677512408e-07 33608.4138040097 -734232.231230357;-0.00044 -1.20749579057035e-07 44676.1519620054 -733641.94792356;-0.0004 -1.20199023188685e-07 55733.7311483156 -732884.840764464;-0.00036 -1.19621135099015e-07 66778.6369647899 -731961.081912707;-0.00032 -1.19016046194791e-07 77808.3578950928 -730870.881423087;-0.00028 -1.18383894068014e-07 88820.3858758011 -729614.487197794;-0.00024 -1.17724822464625e-07 99812.2168667156 -728192.184930039;-0.0002 -1.17038981251822e-07 110781.351420259 -726604.298039093;-0.00016 -1.16326526383985e-07 121725.295249826 -724851.187596741;-0.00012 -1.15587619867205e-07 132641.559796968 -722933.25224518;-8e-05 -1.14822429722452e-07 143527.662797265 -720850.92810637;-4e-05 -1.14031129947367e-07 154381.128844771 -718604.688682862]  x3=[-0.00148 -3.518760494847e-10 714.210166680111 -1454.18503771736;-0.00144 -3.58163591002277e-10 736.056871932115 -1443.250126745;-0.0014 -3.64369689207932e-10 757.736204198925 -1431.98703313989;-0.00136 -3.70492932888451e-10 779.24323378734 -1420.39831803237;-0.00132 -3.76531929671026e-10 800.573070184298 -1408.48661659632;-0.00128 -3.82485306339868e-10 821.720863168945 -1396.25463744993;-0.00124 -3.8835170914846e-10 842.681803915526 -1383.70516203977;-0.0012 -3.94129804127394e-10 863.451126086875 -1370.84104400833;-0.00116 -3.99818277387701e-10 884.024106918237 -1357.66520854511;-0.00112 -4.05415835419615e-10 904.396068291186 -1344.18065172147;-0.00108 -4.10921205386713e-10 924.562377797384 -1330.39043980935;-0.00104 -4.16333135415339e-10 944.518449791957 -1316.29770858402;-0.001 -4.21650394879276e-10 964.259746436229 -1301.90566261103;-0.00096 -4.26871774679575e-10 983.781778729582 -1287.21757451751;-0.00092 -4.31996087519497e-10 1003.08010753022 -1272.23678424804;-0.00088 -4.37022168174493e-10 1022.15034456461 -1256.96669830513;-0.00084 -4.41948873757165e-10 1040.98815342529 -1241.41078897465;-0.0008 -4.4677508397715e-10 1059.58925055698 -1225.57259353622;-0.00076 -4.51499701395862e-10 1077.9494062306 -1209.45571345892;-0.00072 -4.56121651676044e-10 1096.06444550509 -1193.06381358227;-0.00068 -4.60639883826061e-10 1113.93024917672 -1176.40062128296;-0.00064 -4.65053370438885e-10 1131.54275471582 -1159.46992562722;-0.0006 -4.6936110792572e-10 1148.89795719051 -1142.27557650923;-0.00056 -4.73562116744211e-10 1165.9919101774 -1124.82148377571;-0.00052 -4.77655441621181e-10 1182.820726659 -1107.11161633683;-0.00048 -4.8164015176985e-10 1199.38057990758 -1089.15000126371;-0.00044 -4.85515341101495e-10 1215.6677043553 -1070.94072287274;-0.0004 -4.8928012843148e-10 1231.67839645052 -1052.48792179678;-0.00036 -4.92933657679631e-10 1247.40901549993 -1033.79579404368;-0.00032 -4.96475098064905e-10 1262.85598449642 -1014.86859004209;-0.00028 -4.99903644294297e-10 1278.01579093243 -995.710613674976;-0.00024 -5.03218516745963e-10 1292.88498759873 -976.326221300956;-0.0002 -5.06418961646492e-10 1307.46019336821 -956.71982076369;-0.00016 -5.09504251242314e-10 1321.73809396478 -936.895870389583;-0.00012 -5.12473683965181e-10 1335.71544271696 -916.858877973995;-8e-05 -5.15326584591699e-10 1349.38906129619 -896.61339975621;-4e-05 -5.18062304396868e-10 1362.75584043951 -876.164039383385]  x4=[-0.00148 -3.93900603161066e-10 -6436.59844911664 -14213.1446245449;-0.00144 -3.92366065071876e-10 -6221.54551112137 -14308.5859275425;-0.0014 -3.9074230632311e-10 -6005.07784732919 -14400.7735814923;-0.00136 -3.89029696143504e-10 -5787.24468062012 -14489.6866237165;-0.00132 -3.87228623965845e-10 -5568.09554437775 -14575.3048361563;-0.00128 -3.85339499338412e-10 -5347.68027122579 -14657.6087499684;-0.00124 -3.83362751831857e-10 -5126.04898169659 -14736.5796499526;-0.0012 -3.81298830941515e-10 -4903.25207283412 -14812.1995788072;-0.00116 -3.79148205985197e-10 -4679.34020673413 -14884.4513412126;-0.00112 -3.76911365996473e-10 -4454.36429902403 -14953.318507741;-0.00108 -3.74588819613467e-10 -4228.37550728515 -15018.7854185927;-0.00104 -3.72181094963198e-10 -4001.42521941986 -15080.8371871567;-0.001 -3.69688739541486e-10 -3773.5650419665 -15139.459703396;-0.00096 -3.67112320088463e-10 -3544.84678836443 -15194.6396370558;-0.00092 -3.64452422459694e-10 -3315.32246717215 -15246.3644406952;-0.00088 -3.61709651492961e-10 -3085.04427024095 -15294.6223525398;-0.00084 -3.5888463087073e-10 -2854.06456084699 -15339.4023991566;-0.0008 -3.55978002978328e-10 -2622.4358617843 -15380.6943979492;-0.00076 -3.52990428757872e-10 -2390.21084342156 -15418.4889594732;-0.00072 -3.49922587557977e-10 -2157.44231172533 -15452.7774895712;-0.00068 -3.46775176979274e-10 -1924.1831962524 -15483.5521913272;-0.00064 -3.43548912715789e-10 -1690.4865381141 -15510.8060668393;-0.0006 -3.40244528392191e-10 -1456.40547791516 -15534.5329188113;-0.00056 -3.36862775396981e-10 -1221.99324367005 -15554.7273519617;-0.00052 -3.33404422711627e-10 -987.303138699349 -15571.3847742504;-0.00048 -3.29870256735705e-10 -752.388529509048 -15584.5013979235;-0.00044 -3.26261081108082e-10 -517.302833655459 -15594.0742403736;-0.0004 -3.2257771652417e-10 -282.099507598527 -15600.1011248191;-0.00036 -3.18821000549312e-10 -46.8320345462898 -15602.5806807983;-0.00032 -3.14991787428325e-10 188.446087706742 -15601.5123444817;-0.00028 -3.1109094789125e-10 423.681358944517 -15596.8963587996;-0.00024 -3.07119368955358e-10 658.820288694943 -15588.7337733874;-0.0002 -3.03077953723451e-10 893.809408393142 -15577.0264443467;-0.00016 -2.989676211785e-10 1128.59528353976 -15561.7770338231;-0.00012 -2.9478930597468e-10 1363.12452585149 -15542.989009401;-8e-05 -2.90543958224836e-10 1597.34380540112 -15520.6666433153;-4e-05 -2.86232543284436e-10 1831.19986274432 -15494.8150114793]  x5=0.00147040807418893  V1=ones(3,3)  V2=ones(3,3)  I1=ones(3,3)  I2=ones(3,3)  nHarmo=1  Measurements=None  Decoupling=off  VsMag0=0  VrMag0=0  VsAngle0=0  VrAngle0=0  IsMag0=0  IrMag0=0  IsAngle0=0  IrAngle0=0
      settings: AttributesFormatString=\n
  LVD7 : powerlib/Measurements/Three-Phase V-I Measurement  VoltageMeasurement=no  SetLabelV=on  LabelV=Vabc_LVD7  Vpu=on  VpuLL=off  CurrentMeasurement=no  SetLabelI=off  LabelI=A1  Ipu=off  Pbase=100e6  Vbase=735e3  OutputType=Magnitude  PhasorSimulation=off  PSBequivalent=0
  Load Flow Bus1 : powerlib/Measurements/Load Flow Bus  LConnTagsString=a  Phases=single  Connectors=on one side  ID=LG31_13.8  Vbase=13.8e3  Vref=1  Vangle=0  VLF=1  VLFb=1  VLFc=1  angleLF=2.13  angleLFb=0  angleLFc=0
      settings: AttributesFormatString=%<ID>\n%<Vbase>V\n%<VLF>pu\n%<angleLF>deg.
  Load Flow Bus10 : powerlib/Measurements/Load Flow Bus  LConnTagsString=a  Phases=single  Connectors=on one side  ID=LVD7  Vbase=735e3  Vref=1  Vangle=0  VLF=1.053  VLFb=1  VLFc=1  angleLF=-6.263  angleLFb=0  angleLFc=0
      settings: AttributesFormatString=%<ID>\n%<Vbase>V\n%<VLF>pu\n%<angleLF>deg.
  Load Flow Bus11 : powerlib/Measurements/Load Flow Bus  LConnTagsString=a  Phases=single  Connectors=on one side  ID=CHM7  Vbase=735e3  Vref=1  Vangle=0  VLF=1.055  VLFb=1  VLFc=1  angleLF=1.134  angleLFb=0  angleLFc=0
      settings: AttributesFormatString=%<ID>\n%<Vbase>V\n%<VLF>pu\n%<angleLF>deg.
  Load Flow Bus12 : powerlib/Measurements/Load Flow Bus  LConnTagsString=a  Phases=single  Connectors=on one side  ID=LG47  Vbase=735e3  Vref=1  Vangle=0  VLF=1.01  VLFb=1  VLFc=1  angleLF=23.62  angleLFb=0  angleLFc=0
      settings: AttributesFormatString=%<ID>\n%<Vbase>V\n%<VLF>pu\n%<angleLF>deg.
  Load Flow Bus2 : powerlib/Measurements/Load Flow Bus  LConnTagsString=a  Phases=single  Connectors=on one side  ID=LG3_13.8  Vbase=13.8e3  Vref=1  Vangle=0  VLF=1  VLFb=1  VLFc=1  angleLF=1.566  angleLFb=0  angleLFc=0
      settings: AttributesFormatString=%<ID>\n%<Vbase>V\n%<VLF>pu\n%<angleLF>deg.
  Load Flow Bus3 : powerlib/Measurements/Load Flow Bus  LConnTagsString=a  Phases=single  Connectors=on one side  ID=LG4_13.8  Vbase=13.8e3  Vref=1  Vangle=0  VLF=1  VLFb=1  VLFc=1  angleLF=-0.4067  angleLFb=0  angleLFc=0
      settings: AttributesFormatString=%<ID>\n%<Vbase>V\n%<VLF>pu\n%<angleLF>deg.
  Load Flow Bus4 : powerlib/Measurements/Load Flow Bus  LConnTagsString=a  Phases=single  Connectors=on one side  ID=LG2_13.8  Vbase=13.8e3  Vref=1  Vangle=0  VLF=1  VLFb=1  VLFc=1  angleLF=0  angleLFb=0  angleLFc=0
      settings: AttributesFormatString=%<ID>\n%<Vbase>V\n%<VLF>pu\n%<angleLF>deg.
  Load Flow Bus5 : powerlib/Measurements/Load Flow Bus  LConnTagsString=a  Phases=single  Connectors=on one side  ID=LG27  Vbase=735e3  Vref=1  Vangle=0  VLF=1.009  VLFb=1  VLFc=1  angleLF=24.74  angleLFb=0  angleLFc=0
      settings: AttributesFormatString=%<ID>\n%<Vbase>V\n%<VLF>pu\n%<angleLF>deg.
  Load Flow Bus6 : powerlib/Measurements/Load Flow Bus  LConnTagsString=a  Phases=single  Connectors=on one side  ID=LG37  Vbase=735e3  Vref=1  Vangle=0  VLF=0.9995  VLFb=1  VLFc=1  angleLF=26.29  angleLFb=0  angleLFc=0
      settings: AttributesFormatString=%<ID>\n%<Vbase>V\n%<VLF>pu\n%<angleLF>deg.
  Load Flow Bus7 : powerlib/Measurements/Load Flow Bus  LConnTagsString=a  Phases=single  Connectors=on one side  ID=LMO7  Vbase=735e3  Vref=1  Vangle=0  VLF=1.026  VLFb=1  VLFc=1  angleLF=20.27  angleLFb=0  angleLFc=0
      settings: AttributesFormatString=%<ID>\n%<Vbase>V\n%<VLF>pu\n%<angleLF>deg.
  Load Flow Bus8 : powerlib/Measurements/Load Flow Bus  LConnTagsString=a  Phases=single  Connectors=on one side  ID=NEM_ALB7  Vbase=735e3  Vref=1  Vangle=0  VLF=1.043  VLFb=1  VLFc=1  angleLF=12.43  angleLFb=0  angleLFc=0
      settings: AttributesFormatString=%<ID>\n%<Vbase>V\n%<VLF>pu\n%<angleLF>deg.
  Load Flow Bus9 : powerlib/Measurements/Load Flow Bus  LConnTagsString=a  Phases=single  Connectors=on one side  ID=ABI_CHB7  Vbase=735e3  Vref=1  Vangle=0  VLF=1.059  VLFb=1  VLFc=1  angleLF=4.701  angleLFb=0  angleLFc=0
      settings: AttributesFormatString=%<ID>\n%<Vbase>V\n%<VLF>pu\n%<angleLF>deg.
  NEM-ABI 6*236 : powerlib/Elements/Distributed Parameters Line  Phases=3  Length=236  Frequency=60  Resistance="[0.01273  0.3864]/6"  Inductance="[0.9337e-3  4.1264e-3]/6"  Capacitance=[12.74e-9 7.751e-9]*6  x1=[-0.00136 -2.47879393881632e-08 0 0;-0.00132 -2.48404155642182e-08 0 0;-0.00128 -2.48872432439885e-08 0 0;-0.00124 -2.49284117792636e-08 0 0;-0.0012 -2.49639118086736e-08 0 0;-0.00116 -2.49937352598178e-08 0 0;-0.00112 -2.50178753511008e-08 0 0;-0.00108 -2.50363265932739e-08 0 0;-0.00104 -2.50490847906838e-08 0 0;-0.001 -2.50561470422264e-08 0 0;-0.00096 -2.50575117420066e-08 0 0;-0.00092 -2.50531785797034e-08 0 0;-0.00088 -2.50431485406406e-08 0 0;-0.00084 -2.50274239055626e-08 315446.714585289 -699075.660758653;-0.0008 -2.50060082501158e-08 325952.293654903 -694239.522251473;-0.00076 -2.49789064440355e-08 336383.753983833 -689245.5196638;-0.00072 -2.49461246500388e-08 346738.723547957 -684094.788588756;-0.00068 -2.49076703224229e-08 357014.847716494 -678788.500258169;-0.00064 -2.48635522053702e-08 367209.789787425 -673327.861276247;-0.0006 -2.48137803309602e-08 377321.231518841 -667714.113345201;-0.00056 -2.47583660168879e-08 387346.873656088 -661948.532982903;-0.00052 -2.46973218638904e-08 397284.436454604 -656032.431232605;-0.00048 -2.46306617528816e-08 407131.660198305 -649967.153364828;-0.00044 -2.45584008417961e-08 416886.305713431 -643754.078571454;-0.0004 -2.44805555621417e-08 426546.154877712 -637394.619652111;-0.00036 -2.43971436152638e-08 436109.011124751 -630890.222692916;-0.00032 -2.43081839683199e-08 445572.699943504 -624242.366737647;-0.00028 -2.42136968499663e-08 454935.069372746 -617452.563451418;-0.00024 -2.41137037457592e-08 464193.990490405 -610522.356776945;-0.0002 -2.40082273932679e-08 473347.357897664 -603453.322583461;-0.00016 -2.38972917769056e-08 482393.090197712 -596247.068308381;-0.00012 -2.37809221224747e-08 491329.13046903 -588905.232591784;-8e-05 -2.3659144891431e-08 500153.446733121 -581429.484903798;-4e-05 -2.35319877748669e-08 508864.032416564 -573821.525164979]  x2=[-0.00136 -4.44464442615727e-08 0 0;-0.00132 -4.45104540775177e-08 0 0;-0.00128 -4.45643426000472e-08 0 0;-0.00124 -4.46080975753761e-08 0 0;-0.0012 -4.46417090540001e-08 0 0;-0.00116 -4.4665169392959e-08 0 0;-0.00112 -4.46784732575739e-08 0 0;-0.00108 -4.46816176226608e-08 0 0;-0.00104 -4.46746017732182e-08 0 0;-0.001 -4.46574273045897e-08 0 0;-0.00096 -4.46300981221014e-08 0 0;-0.00092 -4.45926204401737e-08 0 0;-0.00088 -4.45450027809082e-08 0 0;-0.00084 -4.44872559721502e-08 177817.551288874 -753238.639327937;-0.0008 -4.44193931450258e-08 189155.500823855 -750471.65516524;-0.00076 -4.43414297309568e-08 200450.438029157 -747534.020219951;-0.00072 -4.42533834581511e-08 211699.794533462 -744426.402484922;-0.00068 -4.4155274347572e-08 222901.012330111 -741149.508605628;-0.00064 -4.40471247083852e-08 234051.544358773 -737704.083719478;-0.0006 -4.39289591328859e-08 245148.855084622 -734090.911286379;-0.00056 -4.38008044909069e-08 256190.421074898 -730310.812910585;-0.00052 -4.36626899237088e-08 267173.731572715 -726364.648153866;-0.00048 -4.3514646837353e-08 278096.289067979 -722253.31434006;-0.00044 -4.33567088955608e-08 288955.60986531 -717977.74635102;-0.0004 -4.3188912012058e-08 299749.224648805 -713538.916414036;-0.00036 -4.3011294342409e-08 310474.679043541 -708937.833880757;-0.00032 -4.28238962753402e-08 321129.534173683 -704175.544997673;-0.00028 -4.26267604235559e-08 331711.367217057 -699253.132668207;-0.00024 -4.24199316140488e-08 342217.771956083 -694171.716206476;-0.0002 -4.22034568779065e-08 352646.359324926 -688932.45108276;-0.00016 -4.19773854396174e-08 362994.757952751 -683536.528660769;-0.00012 -4.17417687058768e-08 373260.614702952 -677985.175926729;-8e-05 -4.14966602538982e-08 383441.595208231 -672279.655210378;-4e-05 -4.12421158192299e-08 393535.38440142 -666421.263897925]  x3=[-0.00136 -2.37530876766971e-10 0 0;-0.00132 -2.4318290472391e-10 0 0;-0.00128 -2.48779634985436e-10 0 0;-0.00124 -2.5431979490335e-10 0 0;-0.0012 -2.59802124693064e-10 0 0;-0.00116 -2.6522537772006e-10 0 0;-0.00112 -2.70588320783369e-10 0 0;-0.00108 -2.75889734395987e-10 0 0;-0.00104 -2.81128413062174e-10 0 0;-0.001 -2.8630316555158e-10 0 0;-0.00096 -2.91412815170112e-10 0 0;-0.00092 -2.96456200027511e-10 0 0;-0.00088 -3.01432173301554e-10 0 0;-0.00084 -3.06339603498828e-10 247.579680310287 -6549.91554752341;-0.0008 -3.11177374712027e-10 346.318244192161 -6545.43753475364;-0.00076 -3.15944386873696e-10 444.978058291828 -6539.47114593392;-0.00072 -3.20639556006378e-10 543.536688218366 -6532.0177377696;-0.00068 -3.25261814469102e-10 641.971722589264 -6523.07900510144;-0.00064 -3.29810111200154e-10 740.260778126575 -6512.65698052015;-0.0006 -3.34283411956081e-10 838.381504746676 -6500.75403390426;-0.00056 -3.38680699546866e-10 936.311590642492 -6487.37287188117;-0.00052 -3.43000974067232e-10 1034.028767357 -6472.51653721174;-0.00048 -3.4724325312401e-10 1131.5108148469 -6456.18840809835;-0.00044 -3.51406572059525e-10 1228.73556653524 -6438.39219741676;-0.0004 -3.55489984170955e-10 1325.68091435191 -6419.1319518718;-0.00036 -3.594925609256e-10 1422.32481376084 -6398.41205107723;-0.00032 -3.63413392172022e-10 1518.64528877273 -6376.2372065598;-0.00028 -3.67251586347008e-10 1614.62043694219 -6352.61246068792;-0.00024 -3.71006270678302e-10 1710.22843434818 -6327.54318552507;-0.0002 -3.74676591383065e-10 1805.44754055659 -6301.03508160825;-0.00016 -3.78261713862021e-10 1900.25610356379 -6273.09417665168;-0.00012 -3.81760822889234e-10 1994.63256472015 -6243.72682417621;-8e-05 -3.85173122797488e-10 2088.55546363227 -6212.93970206452;-4e-05 -3.88497837659209e-10 2182.00344304289 -6180.73981104269]  x4=[-0.00136 -2.75209429216732e-10 0 0;-0.00132 -2.7242841404901e-10 0 0;-0.00128 -2.69585451009256e-10 0 0;-0.00124 -2.66681186562749e-10 0 0;-0.0012 -2.63716281114178e-10 0 0;-0.00116 -2.60691408857473e-10 0 0;-0.00112 -2.57607257622502e-10 0 0;-0.00108 -2.54464528718657e-10 0 0;-0.00104 -2.51263936775391e-10 0 0;-0.001 -2.4800620957971e-10 0 0;-0.00096 -2.44692087910684e-10 0 0;-0.00092 -2.41322325371003e-10 0 0;-0.00088 -2.37897688215607e-10 0 0;-0.00084 -2.34418955177454e-10 5643.35735451297 -27050.4610325484;-0.0008 -2.30886917290436e-10 6050.6126951416 -26962.2880413365;-0.00076 -2.2730237770951e-10 6456.49217862162 -26867.984058337;-0.00072 -2.23666151528065e-10 6860.90351145863 -26767.5705274621;-0.00068 -2.19979065592577e-10 7263.75473400306 -26661.0702818831;-0.00064 -2.16241958314593e-10 7664.95424136092 -26548.5075388372;-0.0006 -2.12455679480079e-10 8064.41080422405 -26429.9078941216;-0.00056 -2.0862109005619e-10 8462.03358961482 -26305.2983162726;-0.00052 -2.04739061995495e-10 8857.73218154077 -26174.7071404338;-0.00048 -2.00810478037697e-10 9251.41660155448 -26038.1640619123;-0.00044 -1.96836231508908e-10 9642.9973292138 -25895.7001294267;-0.0004 -1.92817226118518e-10 10032.3853224381 -25747.3477380466;-0.00036 -1.88754375753693e-10 10419.4920377558 -25593.1406218266;-0.00032 -1.8464860427157e-10 10804.2294504379 -25433.1138461351;-0.00028 -1.80500845289178e-10 11186.5100745146 -25267.3037996807;-0.00024 -1.7631204197114e-10 11566.2469826688 -25095.7481862383;-0.0002 -1.72083146815208e-10 11943.3538260022 -24918.4860160748;-0.00016 -1.67815121435672e-10 12317.7448536707 -24735.5575970792;-0.00012 -1.63508936344697e-10 12689.3349323831 -24547.0045255963;-8e-05 -1.59165570731639e-10 13058.0395657601 -24352.8696769687;-4e-05 -1.54786012240382e-10 13423.7749135476 -24153.1971957867]  x5=0.00133467809810995  V1=ones(3,3)  V2=ones(3,3)  I1=ones(3,3)  I2=ones(3,3)  nHarmo=1  Measurements=None  Decoupling=off  VsMag0=0  VrMag0=0  VsAngle0=0  VrAngle0=0  IsMag0=0  IrMag0=0  IsAngle0=0  IrAngle0=0
      settings: AttributesFormatString=\n
  NEM-ALB 1980 Mvar : powerlib/Elements/Three-Phase Series RLC Load  LConnTagsString=A|B|C  Configuration=Y (grounded)  NominalVoltage=735e3  Vabc=[1e3 1e3 1e3]  Vabcp=[1e3 1e3 1e3]  NominalFrequency=60  UnbalancedPower=off  ActivePower=6600000  InductivePower=1980e6  CapacitivePower=0  Pabc=[10e3 9e3 11e3]  QLabc=[100 90 110]  QCabc=[100 90 110]  Pabcp=[10e3 9e3 11e3]  QLabcp=[100 90 110]  QCabcp=[100 90 110]  Measurements=None  LoadType=constant Z
  NEM-ALB7 : powerlib/Measurements/Three-Phase V-I Measurement  VoltageMeasurement=no  SetLabelV=on  LabelV=Vabc_NEM7  Vpu=on  VpuLL=off  CurrentMeasurement=no  SetLabelI=off  LabelI=A1  Ipu=off  Pbase=100e6  Vbase=735e3  OutputType=Magnitude  PhasorSimulation=off  PSBequivalent=0
  Regulators1 : Subsystem
  Regulators2 : Subsystem
  Regulators3 : Subsystem
  Regulators4 : Subsystem
  MTLa : PMIOPort  Side=Right
  MTLb : PMIOPort  Port=2  Side=Right
  MTLc : PMIOPort  Port=3  Side=Right
  CHM7a : PMIOPort  Port=4  Side=Right
  CHM7b : PMIOPort  Port=5  Side=Right
  CHM7c : PMIOPort  Port=6  Side=Right
  wires:
  Regulators2/1(Pm) -> LG3_2200 MVA/1
  Regulators4/2(Vf) -> LG4-2700 MVA/2
  Regulators4/1(Pm) -> LG4-2700 MVA/1
  Regulators3/2(Vf) -> LG31-200 MVA/2
  Regulators3/1(Pm) -> LG31-200 MVA/1
  Regulators2/2(Vf) -> LG3_2200 MVA/2
  LG3_2200 MVA/1 -> Regulators2/1(m)
  Regulators1/1(Pm) -> LG2_5500 MVA/1
  Regulators1/2(Vf) -> LG2_5500 MVA/2
  LG2_5500 MVA/1 -> Regulators1/1(m)
  LG31-200 MVA/1 -> Regulators3/1(m)
  LG4-2700 MVA/1 -> Regulators4/1(m)
  connections:
  LG2-NENI 3*279km/RConn1 -- "Cs NEM "/LConn1
  LG2-NENI 3*279km/RConn2 -- "Cs NEM "/LConn2
  LG2-NENI 3*279km/RConn3 -- "Cs NEM "/LConn3
  CHB-CHM 3*195km/RConn1 -- "Cs  CHMN "/LConn1
  CHB-CHM 3*195km/RConn2 -- "Cs  CHMN "/LConn2
  CHB-CHM 3*195km/RConn3 -- "Cs  CHMN "/LConn3
  Load Flow Bus2/LConn1 -- 2200 MVA 13.8 kV/735 kV/LConn1 -- LG3_2200 MVA/RConn1 -- 110 MW/LConn1
  2200 MVA 13.8 kV/735 kV/LConn2 -- LG3_2200 MVA/RConn2 -- 110 MW/LConn2
  2200 MVA 13.8 kV/735 kV/LConn3 -- LG3_2200 MVA/RConn3 -- 110 MW/LConn3
  Load Flow Bus1/LConn1 -- 200 MVA 13.8 kV/735 kV/LConn1 -- LG31-200 MVA/RConn1 -- 10 MW/LConn1
  200 MVA 13.8 kV/735 kV/LConn2 -- LG31-200 MVA/RConn2 -- 10 MW/LConn2
  200 MVA 13.8 kV/735 kV/LConn3 -- LG31-200 MVA/RConn3 -- 10 MW/LConn3
  Load Flow Bus6/LConn1 -- 2200 MVA 13.8 kV/735 kV/RConn1 -- 200 MVA 13.8 kV/735 kV/RConn1 -- LG3-LMO 104km/LConn1 -- LG3 660 Mvar/LConn1 -- LG2-LG3 155km/RConn1
  2200 MVA 13.8 kV/735 kV/RConn2 -- LG3 660 Mvar/LConn2 -- LG2-LG3 155km/RConn2 -- 200 MVA 13.8 kV/735 kV/RConn2 -- LG3-LMO 104km/LConn2
  LG3-LMO 104km/RConn1 -- LMO7/RConn1 -- LG4-LMO 3*118km/RConn1 -- LMO 330 Mvar/LConn1
  LG3-LMO 104km/RConn2 -- LMO7/RConn2 -- LG4-LMO 3*118km/RConn2 -- LMO 330 Mvar/LConn2
  LG3-LMO 104km/RConn3 -- LMO7/RConn3 -- LG4-LMO 3*118km/RConn3 -- LMO 330 Mvar/LConn3
  LG4-LMO 3*118km/LConn1 -- LG4 660 Mvar/LConn1 -- 2700 MVA 13.8 kV/735 kV/RConn1 -- Load Flow Bus12/LConn1
  LG4-LMO 3*118km/LConn2 -- 2700 MVA 13.8 kV/735 kV/RConn2 -- LG4 660 Mvar/LConn2
  LG4 660 Mvar/LConn3 -- 2700 MVA 13.8 kV/735 kV/RConn3 -- LG4-LMO 3*118km/LConn3
  Load Flow Bus3/LConn1 -- LG4-2700 MVA/RConn1 -- 2700 MVA 13.8 kV/735 kV/LConn1 -- 135 MW/LConn1
  LG4-2700 MVA/RConn2 -- 2700 MVA 13.8 kV/735 kV/LConn2 -- 135 MW/LConn2
  LG4-2700 MVA/RConn3 -- 2700 MVA 13.8 kV/735 kV/LConn3 -- 135 MW/LConn3
  Load Flow Bus4/LConn1 -- 5500 MVA 13.8 kV/735 kV/LConn1 -- LG2_5500 MVA/RConn1 -- 275 MW/LConn1
  5500 MVA 13.8 kV/735 kV/LConn2 -- LG2_5500 MVA/RConn2 -- 275 MW/LConn2
  LG2_5500 MVA/RConn3 -- 5500 MVA 13.8 kV/735 kV/LConn3 -- 275 MW/LConn3
  5500 MVA 13.8 kV/735 kV/RConn1 -- LG2-NENI 3*279km/LConn1 -- LG2-LG3 155km/LConn1 -- LG2 660 Mvar/LConn1 -- Load Flow Bus5/LConn1
  LG2-LG3 155km/LConn2 -- 5500 MVA 13.8 kV/735 kV/RConn2 -- LG2-NENI 3*279km/LConn2 -- LG2 660 Mvar/LConn2
  LG2-LG3 155km/LConn3 -- 5500 MVA 13.8 kV/735 kV/RConn3 -- LG2-NENI 3*279km/LConn3 -- LG2 660 Mvar/LConn3
  "Cs NEM "/RConn1 -- NEM-ALB7/LConn1 -- Cs ALB/RConn1
  "Cs NEM "/RConn2 -- NEM-ALB7/LConn2 -- Cs ALB/RConn2
  "Cs NEM "/RConn3 -- NEM-ALB7/LConn3 -- Cs ALB/RConn3
  LMO7/LConn1 -- LMO-ALB 3*218km/LConn1
  LMO7/LConn2 -- LMO-ALB 3*218km/LConn2
  Load Flow Bus7/LConn1 -- LMO7/LConn3 -- LMO-ALB 3*218km/LConn3
  Cs ALB/LConn1 -- LMO-ALB 3*218km/RConn1
  Cs ALB/LConn2 -- LMO-ALB 3*218km/RConn2
  Cs ALB/LConn3 -- LMO-ALB 3*218km/RConn3
  200 MVA 13.8 kV/735 kV/RConn3 -- LG3-LMO 104km/LConn3 -- LG3 660 Mvar/LConn3 -- LG2-LG3 155km/RConn3 -- 2200 MVA 13.8 kV/735 kV/RConn3
  Load Flow Bus8/LConn1 -- NEM-ABI 6*236/LConn1 -- NEM-ALB7/RConn1 -- NEM-ALB 1980 Mvar/LConn1
  NEM-ALB 1980 Mvar/LConn2 -- NEM-ALB7/RConn2 -- NEM-ABI 6*236/LConn2
  NEM-ALB 1980 Mvar/LConn3 -- NEM-ALB7/RConn3 -- NEM-ABI 6*236/LConn3
  NEM-ABI 6*236/RConn1 -- "Cs ABI+CHB "/LConn1
  NEM-ABI 6*236/RConn2 -- "Cs ABI+CHB "/LConn2
  NEM-ABI 6*236/RConn3 -- "Cs ABI+CHB "/LConn3
  "Cs ABI+CHB "/RConn1 -- ABI-CHB7/LConn1
  "Cs ABI+CHB "/RConn2 -- ABI-CHB7/LConn2
  "Cs ABI+CHB "/RConn3 -- ABI-CHB7/LConn3
  Load Flow Bus9/LConn1 -- ABI+CHB 1320 Mvar/LConn1 -- CHB-CHM 3*195km/LConn1 -- ABI-CHB 3*271km/LConn1 -- ABI-CHB7/RConn1
  ABI-CHB 3*271km/LConn2 -- ABI-CHB7/RConn2 -- ABI+CHB 1320 Mvar/LConn2 -- CHB-CHM 3*195km/LConn2
  ABI-CHB 3*271km/LConn3 -- ABI-CHB7/RConn3 -- ABI+CHB 1320 Mvar/LConn3 -- CHB-CHM 3*195km/LConn3
  ABI-CHB 3*271km/RConn1 -- "Cs LVDN "/LConn1
  ABI-CHB 3*271km/RConn2 -- "Cs LVDN "/LConn2
  ABI-CHB 3*271km/RConn3 -- "Cs LVDN "/LConn3
  "Cs LVDN "/RConn1 -- LVD7/LConn1
  "Cs LVDN "/RConn2 -- LVD7/LConn2
  "Cs LVDN "/RConn3 -- LVD7/LConn3
  "Cs LVDS "/LConn1 -- LVD 990 Mvar/LConn1 -- Load Flow Bus10/LConn1 -- LVD7/RConn1
  "Cs LVDS "/LConn2 -- LVD7/RConn2 -- LVD 990 Mvar/LConn2
  "Cs LVDS "/LConn3 -- LVD7/RConn3 -- LVD 990 Mvar/LConn3
  "Cs LVDS "/RConn1 -- LVD-MTL 3*260km/LConn1
  "Cs LVDS "/RConn2 -- LVD-MTL 3*260km/LConn2
  "Cs LVDS "/RConn3 -- LVD-MTL 3*260km/LConn3
  MTLa/RConn1 -- LVD-MTL 3*260km/RConn1
  MTLb/RConn1 -- LVD-MTL 3*260km/RConn2
  MTLc/RConn1 -- LVD-MTL 3*260km/RConn3
  "Cs  CHMN "/RConn1 -- CHM7/LConn1
  "Cs  CHMN "/RConn2 -- CHM7/LConn2
  "Cs  CHMN "/RConn3 -- CHM7/LConn3
  CHM 1320Mvar/LConn2 -- CHM7/RConn2 -- CHM7b/RConn1
  Load Flow Bus11/LConn1 -- CHM 1320Mvar/LConn3 -- CHM7c/RConn1 -- CHM7/RConn3
  CHM7a/RConn1 -- CHM 1320Mvar/LConn1 -- CHM7/RConn1
